simulink model "mdt_snap_10ch_daq"  (R2018a)
settings: Solver=VariableStepAuto  StartTime=0.0  StopTime=2000  RelTol=1e-3
libraries: xbsIndex_r4 x1064, xps_library x6, casper_library_misc x6, simulink x1
(part 1 of 12)
settings Model: Creator=aragorn  LastModifiedBy=aragorn

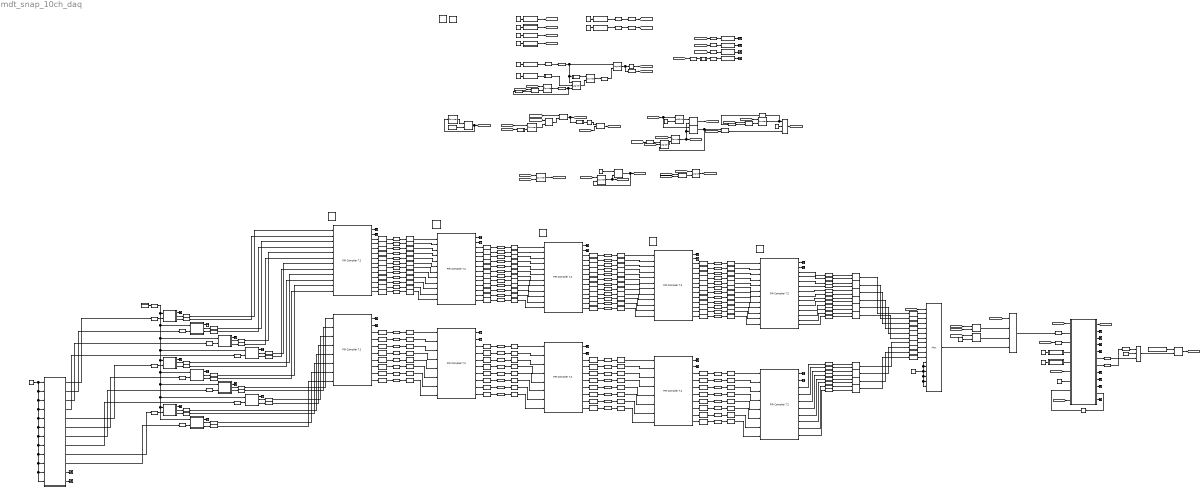
== system mdt_snap_10ch_daq ==
  note: Circuit to decimate FPGA clock. Decimation factor M stored as a constant.
      | Output: a high pulse 1 clock width at the last cycle of every M cycles.
      | Note: initial value of counter is 1; number of bits for counter and constant should be same or sufficient to accomodate value M.
  note: 1/1000 x FPGA clock period.
  note: stationIdx: MDT station ID
      |
      | snapIdx: SNAP board ID in the station
      |
      | Nelements: number of elements in instrument, i.e. number of analogue channels that the SNAP board need to process: at most 10.
      |
      | SperElement: number of samples taken per analogue channel to fit into 1 UDP packet.
      |
      | PktLimit: number of packets to acquire in one go and stored in bram.
  note: ch_valid is set to high after each decimated clk, during {0, Nelements-1}.
      | ch_last is 1 on clock cycle when counter = Nelements-1.
  note: Circuit counts the number of samples per channel being added to the current packet. Once the number of samples is equal to SperElement the end_pkt signal will be high at the last sample of the last batch in the packet. Then, on the next clock the new_pkt signal is high.
      | Note that the new_pkt signal is also set to high when enable pkt is set to 1 at the beginning of acquisition.
  note: Circuit to enable input of the header to the 10gbe block.
  note: Circuit to enable data input to the 10gbe block.
  note: Circuit to count packets for the duration of observation.
  note: 2^32 - 1 = 4294967295
  note: When enable_daq is set to 1, the packetiser will start working when the trigger for the 1PPS is received via 10 GbE from the script.
  note: Byte-swapping to obtain Little-Endian at output. Also concatenates the two samples to form a pair.
  note: SNAP FPGA is clocked at 250 MHz and ADC samples at 250 MSps. Therefore, we obtain 1 sample per analogue channel digitised.
      |
      | DDC mixer works with LO at 77.4 MHz and outputs complex samples.
      |
      | The 5-stage filter cuts out the relevant 250 kHz bandwidth centered at 327.4 MHz and decimates the sampling frequency to 250 kSps.
      |
      | The samples are then input sequentially to the 10gbe block. The packetiser circuit also includes a header with each packet.
  note: LPF with cut-off at 125 kHz and roll-off up to 250 kHz at -80 dB
      | Kaiser window with 82 taps.
      | Decimation factor: 4
      | Output at 500 kSps
  note: Quadrature mixing with LO at frequency = (10145/32768) x 250 MHz
      | = 77.4 MHz
  note: LPF with cut-off at 140 kHz and roll-off up to ~5 MHz at -98 dB
      | Kaiser window with 66 taps.
      | Decimation factor: 5
      | Output at 10 MSps
  note: LPF with cut-off at 130 kHz and roll-off up to 1 MHz at -89 dB
      | Kaiser window with 66 taps.
      | Decimation factor: 5
      | Output at 2 MSps
  note: LPF with cut-off at 123 kHz and roll-off up to 126 kHz at -72 dB
      | Kaiser window with 710 taps.
      | Decimation factor: 2
      | Output at 250 kSps
  note: LPF with cut-off at 140 kHz and roll-off up to ~25 MHz at -100 dB
      | Kaiser window with 66 taps.
      | Decimation factor: 5
      | Output at 50 MSps
  note: ADC2
      |
      | SMATP9
      | SMATP10
      | SMATP11
      | SMATP12
  note: SMATP1 -- SMATP6
  note: Decimation Filter Stage 1
  note: Digital Down-Conversion
  note: ADC
  note: SMATP7 -- SMATP10
  note: SMATP1 -- SMATP6
  note: SMATP7 -- SMATP10
  note: Decimation Filter Stage 2
  note: SMATP1 -- SMATP6
  note: SMATP7 -- SMATP10
  note: Decimation Filter Stage 3
  note: SMATP7 -- SMATP10
  note: SMATP1 -- SMATP6
  note: Decimation Filter Stage 4
  note: SMATP7 -- SMATP10
  note: SMATP1 -- SMATP6
  note: Decimation Filter Stage 5
  note: Byte-Swapping
  note: Packetisation
  note: Byte-swapping
      | for header
  note: LED 0 : data acquisition enabled
      |
      | LED 1 : 10 GbE port 0 is up and connected
      |
      | LED 2 : UDP packet being constructed
      |
      | LED 3 : end of current UDP packet
  note: ADC1
      |
      | SMATP5
      | SMATP6
      | SMATP7
      | SMATP8
  note: ADC0
      |
      | SMATP1
      | SMATP2
      | SMATP3
      | SMATP4
  note: Send data out in UDP packets
  note: Header
  note: Receive signal to start acquisition
  note: mdt_snap_10ch_daq.slx
      |
      | Copyright (c) 2020 Nitish Ragoomundun, Mauritius
      |
      | Permission is hereby granted, free of charge, to any person obtaining a copy
      | of this software and associated documentation files (the "Software"), to deal
      | in the Software without restriction, including without limitation the rights
      | to use, copy, modify, merge, publish, distribute, sublicense, and/or sell
      | copies of the Software, and to permit persons to whom the Software is
      | furnished to do so, subject to the following conditions:
      |
      | The above copyright notice and this permission notice shall be included in all
      | copies or substantial portions of the Software.
      |
      | THE SOFTWARE IS PROVIDED "AS IS", WITHOUT WARRANTY OF ANY KIND, EXPRESS OR
      | IMPLIED, INCLUDING BUT NOT LIMITED TO THE WARRANTIES OF MERCHANTABILITY,
      | FITNESS FOR A PARTICULAR PURPOSE AND NONINFRINGEMENT. IN NO EVENT SHALL THE
      | AUTHORS OR COPYRIGHT HOLDERS BE LIABLE FOR ANY CLAIM, DAMAGES OR OTHER
      | LIABILITY, WHETHER IN AN ACTION OF CONTRACT, TORT OR OTHERWISE, ARISING FROM,
      | OUT OF OR IN CONNECTION WITH THE SOFTWARE OR THE USE OR OTHER DEALINGS IN THE
      | SOFTWARE.
  " System Generator" : xbsIndex_r4/ System Generator  Tag=genX  xilinxfamily=kintex7  part=xc7k160t  speed=-2  package=ffg676  synthesis_tool=XST  clock_wrapper=Clock Enables  directory=/home/aragorn/Documents/SNAP/MDT_SNAP_DAQ/mdt_snap_10ch_daq/sysgen  proj_type=Vivado  Synth_file=Vivado Synthesis Defaults  Impl_file=Vivado Implementation Defaults  testbench=off  simulink_period=1  sysclk_period=4  dcm_input_clock_period=10  incr_netlist=off  trim_vbits=Everywhere in SubSystem  dbl_ovrd=According to Block Masks  core_generation=According to Block Masks  run_coregen=off  deprecated_control=off  eval_field=0  block_type=sysgen
  AddSub1 : xbsIndex_r4/AddSub  mode=Subtraction  use_carryin=off  use_carryout=off  en=off  latency=0  precision=User Defined  arith_type=Unsigned  n_bits=4  bin_pt=0  quantization=Truncate  overflow=Wrap  use_behavioral_HDL=off  hw_selection=Fabric  pipelined=off  dbl_ovrd=off  block_type=addsub
  Band-Limited White Noise : simulink/Sources/Band-Limited White Noise  Cov=[0.1]  Ts=1.0  seed=[23341]
  BitBasher{1..12} (12 alike) : xbsIndex_r4/BitBasher  bitexpr=c = {a[7:0], a[15:8], a[23:16], a[31:24], b[7:0], b[15:8], b[23:16], b[31:24]}  display_expr=off  sr_1=c  arith_type1=Unsigned  bin_pt1=0  sr_2=2  arith_type2=Unsigned  bin_pt2=0  sr_3=3  arith_type3=Unsigned  bin_pt3=0  sr_4=4  arith_type4=Unsigned  bin_pt4=0  dbl_ovrd=off  block_type=bitbasher
  Constant : xbsIndex_r4/Constant  const=1000  gui_display_data_type=Fixed-point  arith_type=Unsigned  n_bits=10  bin_pt=0  preci_type=Single  exp_width=8  frac_width=24  explicit_period=on  period=1  equ=P=C  opselect=C  inp2=PCIN>>17  opr=+  inp1=P  carry=CIN  dbl_ovrd=off  block_type=constant
  Constant{1..2,4,8,105..106,114} (7 alike) : Constant  Value=0
  Constant107 : xbsIndex_r4/Constant  const=0  gui_display_data_type=Fixed-point  arith_type=Unsigned  n_bits=32  bin_pt=0  preci_type=Single  exp_width=8  frac_width=24  explicit_period=on  period=1  equ=P=C  opselect=C  inp2=PCIN>>17  opr=+  inp1=P  carry=CIN  dbl_ovrd=off  block_type=constant
  Constant108 : Constant  Value=3
  Constant109 : Constant  Value=8
  Constant110 : xbsIndex_r4/Constant  const=1  gui_display_data_type=Fixed-point  arith_type=Unsigned  n_bits=1  bin_pt=0  preci_type=Single  exp_width=8  frac_width=24  explicit_period=on  period=1  equ=P=C  opselect=C  inp2=PCIN>>17  opr=+  inp1=P  carry=CIN  dbl_ovrd=off  block_type=constant
  Constant111 : xbsIndex_r4/Constant  const=0  gui_display_data_type=Boolean  arith_type=Boolean  n_bits=1  bin_pt=0  preci_type=Single  exp_width=8  frac_width=24  explicit_period=on  period=1  equ=P=C  opselect=C  inp2=PCIN>>17  opr=+  inp1=P  carry=CIN  dbl_ovrd=off  block_type=constant
  Constant3 : xbsIndex_r4/Constant  const=2  gui_display_data_type=Fixed-point  arith_type=Unsigned  n_bits=2  bin_pt=0  preci_type=Single  exp_width=8  frac_width=24  explicit_period=on  period=1  equ=P=C  opselect=C  inp2=PCIN>>17  opr=+  inp1=P  carry=CIN  dbl_ovrd=off  block_type=constant
  Constant5 : xbsIndex_r4/Constant  const=0  gui_display_data_type=Fixed-point  arith_type=Unsigned  n_bits=64  bin_pt=0  preci_type=Single  exp_width=8  frac_width=24  explicit_period=on  period=1  equ=P=C  opselect=C  inp2=PCIN>>17  opr=+  inp1=P  carry=CIN  dbl_ovrd=off  block_type=constant
  Constant6 : xbsIndex_r4/Constant  const=12012006508534266765  gui_display_data_type=Fixed-point  arith_type=Unsigned  n_bits=64  bin_pt=0  preci_type=Single  exp_width=8  frac_width=24  explicit_period=on  period=1  equ=P=C  opselect=C  inp2=PCIN>>17  opr=+  inp1=P  carry=CIN  dbl_ovrd=off  block_type=constant
  Constant7 : xbsIndex_r4/Constant  const=0  gui_display_data_type=Fixed-point  arith_type=Unsigned  n_bits=64  bin_pt=0  preci_type=Single  exp_width=8  frac_width=24  explicit_period=on  period=1  equ=P=C  opselect=C  inp2=PCIN>>17  opr=+  inp1=P  carry=CIN  dbl_ovrd=off  block_type=constant
  Constant9 : xbsIndex_r4/Constant  const=1  gui_display_data_type=Boolean  arith_type=Boolean  n_bits=16  bin_pt=14  preci_type=Single  exp_width=8  frac_width=24  explicit_period=on  period=1  equ=P=C  opselect=C  inp2=PCIN>>17  opr=+  inp1=P  carry=CIN  dbl_ovrd=off  block_type=constant
  Convert{,2,4,6,8..9,25..34,39..42} (20 alike) : xbsIndex_r4/Convert  gui_display_data_type=Fixed-point  arith_type="Signed  (2's comp)"  n_bits=16  bin_pt=12  float_type=Single  exp_bits=8  fraction_bits=24  quantization="Round  (unbiased: +/- Inf)"  overflow=Wrap  en=off  latency=1  pipeline=on  dbl_ovrd=off  block_type=convert
  Convert1 : xbsIndex_r4/Convert  gui_display_data_type=Boolean  arith_type=Boolean  n_bits=16  bin_pt=14  float_type=Single  exp_bits=8  fraction_bits=24  quantization=Truncate  overflow=Wrap  en=off  latency=0  pipeline=off  dbl_ovrd=off  block_type=convert
  Convert{10..15,43..56} (20 alike) : xbsIndex_r4/Convert  gui_display_data_type=Fixed-point  arith_type="Signed  (2's comp)"  n_bits=16  bin_pt=10  float_type=Single  exp_bits=8  fraction_bits=24  quantization="Round  (unbiased: +/- Inf)"  overflow=Wrap  en=off  latency=1  pipeline=on  dbl_ovrd=off  block_type=convert
  Convert{3,16..20,61..73,78} (20 alike) : xbsIndex_r4/Convert  gui_display_data_type=Fixed-point  arith_type="Signed  (2's comp)"  n_bits=16  bin_pt=8  float_type=Single  exp_bits=8  fraction_bits=24  quantization="Round  (unbiased: +/- Inf)"  overflow=Wrap  en=off  latency=1  pipeline=on  dbl_ovrd=off  block_type=convert
  Convert{5,7,21..24,79..90,95..96} (20 alike) : xbsIndex_r4/Convert  gui_display_data_type=Fixed-point  arith_type="Signed  (2's comp)"  n_bits=16  bin_pt=6  float_type=Single  exp_bits=8  fraction_bits=24  quantization="Round  (unbiased: +/- Inf)"  overflow=Wrap  en=off  latency=1  pipeline=on  dbl_ovrd=off  block_type=convert
  Counter1 : xbsIndex_r4/Counter  cnt_type=Free Running  cnt_to=Inf  operation=Up  start_count=0  cnt_by_val=1  arith_type=Unsigned  n_bits=2  bin_pt=0  load_pin=off  rst=on  en=on  explicit_period=on  period=1  use_behavioral_HDL=off  implementation=Fabric  dbl_ovrd=off  block_type=counter
  Counter10 : xbsIndex_r4/Counter  cnt_type=Free Running  cnt_to=Inf  operation=Up  start_count=0  cnt_by_val=1  arith_type=Unsigned  n_bits=16  bin_pt=0  load_pin=off  rst=on  en=on  explicit_period=on  period=1  use_behavioral_HDL=off  implementation=Fabric  dbl_ovrd=off  block_type=counter
  Counter11 : xbsIndex_r4/Counter  cnt_type=Free Running  cnt_to=Inf  operation=Up  start_count=0  cnt_by_val=1  arith_type=Unsigned  n_bits=1  bin_pt=0  load_pin=off  rst=on  en=on  explicit_period=on  period=1  use_behavioral_HDL=off  implementation=Fabric  dbl_ovrd=off  block_type=counter
  Counter2 : xbsIndex_r4/Counter  cnt_type=Free Running  cnt_to=Inf  operation=Up  start_count=0  cnt_by_val=1  arith_type=Unsigned  n_bits=32  bin_pt=0  load_pin=off  rst=on  en=on  explicit_period=on  period=1  use_behavioral_HDL=off  implementation=Fabric  dbl_ovrd=off  block_type=counter
  Counter3 : xbsIndex_r4/Counter  cnt_type=Free Running  cnt_to=Inf  operation=Up  start_count=1  cnt_by_val=1  arith_type=Unsigned  n_bits=10  bin_pt=0  load_pin=off  rst=on  en=off  explicit_period=on  period=1  use_behavioral_HDL=off  implementation=Fabric  dbl_ovrd=off  block_type=counter
  Counter4 : xbsIndex_r4/Counter  cnt_type=Free Running  cnt_to=Inf  operation=Up  start_count=0  cnt_by_val=1  arith_type=Unsigned  n_bits=2  bin_pt=0  load_pin=off  rst=on  en=on  explicit_period=on  period=1  use_behavioral_HDL=off  implementation=Fabric  dbl_ovrd=off  block_type=counter
  Counter6 : xbsIndex_r4/Counter  cnt_type=Free Running  cnt_to=Inf  operation=Up  start_count=0  cnt_by_val=1  arith_type=Unsigned  n_bits=2  bin_pt=0  load_pin=off  rst=on  en=on  explicit_period=on  period=1  use_behavioral_HDL=off  implementation=Fabric  dbl_ovrd=off  block_type=counter
  Counter7 : xbsIndex_r4/Counter  cnt_type=Free Running  cnt_to=Inf  operation=Up  start_count=0  cnt_by_val=1  arith_type=Unsigned  n_bits=4  bin_pt=0  load_pin=off  rst=on  en=on  explicit_period=on  period=1  use_behavioral_HDL=off  implementation=Fabric  dbl_ovrd=off  block_type=counter
  Delay1 : xbsIndex_r4/Delay  rst=off  infoeditControl=Selection of Reset will increase slice count due to use of real FFs and instead of SRLs  en=off  latency=1  reg_retiming=off  dbl_ovrd=off  block_type=delay
  Delay2 : xbsIndex_r4/Delay  rst=off  infoeditControl=Selection of Reset will increase slice count due to use of real FFs and instead of SRLs  en=off  latency=1  reg_retiming=off  dbl_ovrd=off  block_type=delay
  Delay4 : xbsIndex_r4/Delay  rst=off  infoeditControl=Selection of Reset will increase slice count due to use of real FFs and instead of SRLs  en=off  latency=1  reg_retiming=off  dbl_ovrd=off  block_type=delay
  Inverter1 : xbsIndex_r4/Inverter  en=off  latency=0  dbl_ovrd=off  block_type=inv
  Inverter2 : xbsIndex_r4/Inverter  en=off  latency=0  dbl_ovrd=off  block_type=inv
  Inverter3 : xbsIndex_r4/Inverter  en=off  latency=0  dbl_ovrd=off  block_type=inv
  Logical1 : xbsIndex_r4/Logical  logical_function=AND  inputs=3  en=off  latency=0  precision=User Defined  arith_type=Boolean  n_bits=1  bin_pt=0  align_bp=on  dbl_ovrd=off  block_type=logical
  Logical10 : xbsIndex_r4/Logical  logical_function=OR  inputs=2  en=off  latency=0  precision=User Defined  arith_type=Boolean  n_bits=1  bin_pt=0  align_bp=on  dbl_ovrd=off  block_type=logical
  Logical{2..3,6..9} (6 alike) : xbsIndex_r4/Logical  logical_function=AND  inputs=2  en=off  latency=0  precision=User Defined  arith_type=Boolean  n_bits=1  bin_pt=0  align_bp=on  dbl_ovrd=off  block_type=logical
  Logical4 : xbsIndex_r4/Logical  logical_function=OR  inputs=2  en=off  latency=0  precision=User Defined  arith_type=Boolean  n_bits=1  bin_pt=0  align_bp=on  dbl_ovrd=off  block_type=logical
  Logical5 : xbsIndex_r4/Logical  logical_function=AND  inputs=3  en=off  latency=0  precision=User Defined  arith_type=Boolean  n_bits=1  bin_pt=0  align_bp=on  dbl_ovrd=off  block_type=logical
  Mux1 : xbsIndex_r4/Mux  inputs=2  en=off  latency=0  precision=Full  arith_type=Unsigned  n_bits=16  bin_pt=14  quantization=Truncate  overflow=Wrap  dbl_ovrd=off  block_type=mux
  Mux3 : xbsIndex_r4/Mux  inputs=16  en=off  latency=0  precision=Full  arith_type=Unsigned  n_bits=16  bin_pt=14  quantization=Truncate  overflow=Wrap  dbl_ovrd=off  block_type=mux
  Mux4 : xbsIndex_r4/Mux  inputs=3  en=off  latency=0  precision=Full  arith_type=Unsigned  n_bits=16  bin_pt=14  quantization=Truncate  overflow=Wrap  dbl_ovrd=off  block_type=mux
  Mux5 : xbsIndex_r4/Mux  inputs=2  en=off  latency=0  precision=Full  arith_type=Unsigned  n_bits=16  bin_pt=14  quantization=Truncate  overflow=Wrap  dbl_ovrd=off  block_type=mux
  Nelements : Subsystem  Tag=xps:sw_reg  AncestorBlock=xps_library/Memory/software_register  mask(swreg){io_dir=From Processor, io_delay=0, init_val=0, sample_period=1, names=reg, bitwidths=32, bin_pts=0, arith_types=0, sim_port=on, show_format=on}
      mask prompts: io_dir "I/O direction"; io_delay "I/O delay"; init_val "Initial Value"; sample_period "Sample period"; names "Bitfield names [msb...lsb]"; bitwidths "Bitfield widths"; bin_pts "Bitfield binary pts"; arith_types "Bitfield types, ufix=0, fix=1, bool=2"; sim_port "Provide sim input/output?"; show_format "Print format string?"
      mask help: A 32-bit software-accessible register. Can be divided into bitfields of varying widths and types using the fields in the block mask.
      mask init:
      | swreg_init(gcb)
      settings: AttributesFormatString=1input:uf32.0 = 32 bits
      mask TypeOptions io_dir: To Processor | From Processor
      mask Callback io_dir:
      | mask_enables = get_param(gcb, 'MaskEnables');
      | mask_names = get_param(gcb, 'MaskNames');
      | if strcmp(get_param(gcb, 'io_dir'), 'To Processor'),
      |     mask_enables{ismember(mask_names, 'sample_period')} = 'off';
      | else
      |     mask_enables{ismember(mask_names, 'sample_period')} = 'on';
      | end
      | set_param(gcb, 'MaskEnables', mask_enables);
      mask DialogControl ParameterTabVar0 Prompt: Setup
  Pulse Generator : DiscretePulseGenerator  PulseType=Time based  Period=1  PulseWidth=20
  Register{1..32,38..42,44..48,55} (43 alike) : xbsIndex_r4/Register  init=0  rst=off  en=off  dbl_ovrd=off  block_type=register
  Reinterpret{1..6,25,107..115,120..124} (21 alike) : xbsIndex_r4/Reinterpret  force_arith_type=on  arith_type=Unsigned  force_bin_pt=on  bin_pt=0  block_type=reinterpret
  Reinterpret{7..11,36,89..99,101,103..104} (20 alike) : xbsIndex_r4/Reinterpret  force_arith_type=off  arith_type=Unsigned  force_bin_pt=on  bin_pt=22  block_type=reinterpret
  Reinterpret{12..24,29..31,33..34,51..52} (20 alike) : xbsIndex_r4/Reinterpret  force_arith_type=off  arith_type=Unsigned  force_bin_pt=on  bin_pt=28  block_type=reinterpret
  Reinterpret{32,45..49,71..84} (20 alike) : xbsIndex_r4/Reinterpret  force_arith_type=off  arith_type=Unsigned  force_bin_pt=on  bin_pt=24  block_type=reinterpret
  Reinterpret{37,40..44,53..66} (20 alike) : xbsIndex_r4/Reinterpret  force_arith_type=off  arith_type=Unsigned  force_bin_pt=on  bin_pt=26  block_type=reinterpret
  Relational{1..2,10,13} (4 alike) : xbsIndex_r4/Relational  mode=a=b  op_type=Bool  en=off  latency=0  dbl_ovrd=off  block_type=relational
  Relational11 : xbsIndex_r4/Relational  mode=a>b  op_type=Bool  en=off  latency=0  dbl_ovrd=off  block_type=relational
  Relational12 : xbsIndex_r4/Relational  mode=a>b  op_type=Bool  en=off  latency=0  dbl_ovrd=off  block_type=relational
  SNAP : xps_library/Platforms/SNAP  Tag=xps:xsg  hw_sys=SNAP:xc7k160t  clk_src=adc0_clk  clk_rate=250  use_microblaze=off  sample_period=1  synthesis_tool=XST
      settings: SourceProductName=CASPER XPS Blockset
  Shift{,1..32,37..54,59..72,76,78..90,95} (80 alike) : xbsIndex_r4/Shift  shift_dir=Left  shift_bits=2  en=off  latency=1  precision=Full  arith_type="Signed  (2's comp)"  n_bits=16  bin_pt=14  quantization=Truncate  overflow=Wrap  dbl_ovrd=off  block_type=shift
  Slice{1..5} (5 alike) : xbsIndex_r4/Slice  nbits=1  boolean_output=on  mode=Lower Bit Location + Width  bit1=0  base1=MSB of Input  bit0=0  base0=LSB of Input  dbl_ovrd=off  block_type=slice
  SperElement : Subsystem  Tag=xps:sw_reg  AncestorBlock=xps_library/Memory/software_register  mask(swreg){io_dir=From Processor, io_delay=0, init_val=0, sample_period=1, names=reg, bitwidths=32, bin_pts=0, arith_types=0, sim_port=on, show_format=on}
      mask prompts: io_dir "I/O direction"; io_delay "I/O delay"; init_val "Initial Value"; sample_period "Sample period"; names "Bitfield names [msb...lsb]"; bitwidths "Bitfield widths"; bin_pts "Bitfield binary pts"; arith_types "Bitfield types, ufix=0, fix=1, bool=2"; sim_port "Provide sim input/output?"; show_format "Print format string?"
      mask help: A 32-bit software-accessible register. Can be divided into bitfields of varying widths and types using the fields in the block mask.
      mask init:
      | swreg_init(gcb)
      settings: AttributesFormatString=1input:uf32.0 = 32 bits
      mask TypeOptions io_dir: To Processor | From Processor
      mask Callback io_dir:
      | mask_enables = get_param(gcb, 'MaskEnables');
      | mask_names = get_param(gcb, 'MaskNames');
      | if strcmp(get_param(gcb, 'io_dir'), 'To Processor'),
      |     mask_enables{ismember(mask_names, 'sample_period')} = 'off';
      | else
      |     mask_enables{ismember(mask_names, 'sample_period')} = 'on';
      | end
      | set_param(gcb, 'MaskEnables', mask_enables);
      mask DialogControl ParameterTabVar0 Prompt: Setup
  Stage1_ch1-6 : xbsIndex_r4/FIR Compiler 7.2   coefficientvector=[-0.000002449538004038990423916243369117, -0.000005500349966184503970535908667915, -0.000005285271766498275070804251096756, 0.000005201883925181383781951010430999, 0.000035996819259535929092820583097278, 0.000098266946066012054311622492264177, 0.000200426952388683672721253481441294, 0.000342426747931809155513910303270108, 0.000509090254199270376977981555910446, 0.000664151073096023460660963788626531, 0.000747226168430985336448013622856478, 0.000676147634572773440636561659289327, 0.000356634720256595130240262481180479, -0.000299853285296282356942043634262518, -0.001351005061725356337642978132862481, -0.002794317437538150830644845257211272, -0.004538578190165965149660554089905417, -0.006382626815274574164082999061520240, -0.008008145384657154586260929818308795, -0.008992087975882372477554049794434831, -0.008841716737080985988317394230762147, -0.007051359492092778950833587003899083, -0.003175552799073219373965359935141350, 0.003090960705163858963928635859019777, 0.011838921151523604941013800839755276, 0.022889486804945475412198518938566849, 0.035770526437351526927166389668855117, 0.049732447110816674351596589076507370, 0.063805828276941325971627350099879549, 0.076896215021160799207855518488941015, 0.087904748254232167870014791333233006, 0.095858174396951711937475693048327229, 0.100029250702665883920872147427871823, 0.100029250702665883920872147427871823, 0.095858174396951711937475693048327229, 0.087904748254232167870014791333233006, 0.076896215021160799207855518488941015, 0.063805828276941325971627350099879549, 0.049732447110816674351596589076507370, 0.035770526437351526927166389668855117, 0.022889486804945475412198518938566849, 0.011838921151523604941013800839755276, 0.003090960705163858963928635859019777, -0.003175552799073219373965359935141350, -0.007051359492092778950833587003899083, -0.008841716737080985988317394230762147, -0.008992087975882372477554049794434831, -0.008008145384657154586260929818308795, -0.006382626815274574164082999061520240, -0.004538578190165965149660554089905417, -0.002794317437538150830644845257211272, -0.001351005061725356337642978132862481, -0.000299853285296282356942043634262518, 0.000356634720256595130240262481180479, 0.000676147634572773440636561659289327, 0.000747226168430985336448013622856478, 0.000664151073096023460660963788626531, 0.000509090254199270376977981555910446, 0.000342426747931809155513910303270108, 0.000200426952388683672721253481441294, 0.000098266946066012054311622492264177, 0.000035996819259535929092820583097278, 0.000005201883925181383781951010430999, -0.000005285271766498275070804251096756, -0.000005500349966184503970535908667915, -0.000002449538004038990423916243369117]  coefficient_sets=1  coefficient_reload=off  filter_type=Decimation  rate_change_type=Integer  interpolation_rate=1  decimation_rate=5  zero_pack_factor=1  channel_sequence=Basic  number_channels=1  pattern_list='P4-0,P4-1,P4-2,P4-3,P4-4'  number_paths=12  ratespecification=Maximum_Possible  sampleperiod=1  hardwareoversamplingrate=1  coefficient_sign=Signed  quantization=Maximize_Dynamic_Range  coefficient_width=25  bestprecision=off  coefficient_fractional_bits=24  coefficient_structure=Inferred  output_rounding_mode=Symmetric_Rounding_to_Infinity  output_width=32  filter_architecture=Systolic_Multiply_Accumulate  optimization_goal=Area  optimization_list='None'  data_buffer_type=Automatic  coefficient_buffer_type=Automatic  input_buffer_type=Automatic  output_buffer_type=Automatic  preference_for_other_storage=Automatic  multi_column_support=Automatic  columnconfig='7'  inter_column_pipe_length=4  data_has_tlast=Not_Required  m_data_has_tready=off  s_data_has_fifo=off  s_data_has_tuser=Not_Required  m_data_has_tuser=Not_Required  s_config_sync_mode=On_Vector  s_config_method=Single  num_reload_slots=1  has_aclken=off  has_aresetn=off  infoeditControl=ARESETn must be asserted for a minimum of 2 cycles  reset_data_vector=on  trim_axipin_name=on  simulation_type=hybrid_sim  simulation_model=sysgen:xfirv7_2_cmodel  data_path_portlist={ 's_axis_data_tdata', 'm_axis_data_tdata' }  passband_min=0.0  passband_max=0.5  stopband_min=0.5  stopband_max=1.0  filter_selection=1  gui_behaviour='Sysgen_GUI'  data_sign=Signed  data_width=16  data_fractional_bits=0  data_tuser_width=1  wrapper_available=true  ip_wrap_arbitrary_binary_point=true  ip_name=FIR Compiler  ip_version=7.2  dsptool_ready=true  ipcore_usecache=true  ipcore_useipmodelcache=true  port_translation_map={ 'aclken' => 'en', 'aresetn' => 'rst' }  run_core_at_system_period=true  ipcore_xco_need_fpga_part=true  block_type=fir_compiler_v7_2
      settings: infoedit=Maximum Possible : Maximizes oversampling rate. Abstracted input handshake (no s_data_tvalid) and automatic rate propagation.<br>Hardware Oversampling Rate : Specifies oversampling rate relative to the input sample period. Abstracted input handshake (no s_data_tvalid) and automatic rate propagation.<br>Input/Output Sample Period : Specifies absolute oversampling rate. No input handshake abstraction (exposes s_data_tvalid) and no rate propagation.
  Stage1_ch7-10 : xbsIndex_r4/FIR Compiler 7.2   coefficientvector=[-0.000002449538004038990423916243369117, -0.000005500349966184503970535908667915, -0.000005285271766498275070804251096756, 0.000005201883925181383781951010430999, 0.000035996819259535929092820583097278, 0.000098266946066012054311622492264177, 0.000200426952388683672721253481441294, 0.000342426747931809155513910303270108, 0.000509090254199270376977981555910446, 0.000664151073096023460660963788626531, 0.000747226168430985336448013622856478, 0.000676147634572773440636561659289327, 0.000356634720256595130240262481180479, -0.000299853285296282356942043634262518, -0.001351005061725356337642978132862481, -0.002794317437538150830644845257211272, -0.004538578190165965149660554089905417, -0.006382626815274574164082999061520240, -0.008008145384657154586260929818308795, -0.008992087975882372477554049794434831, -0.008841716737080985988317394230762147, -0.007051359492092778950833587003899083, -0.003175552799073219373965359935141350, 0.003090960705163858963928635859019777, 0.011838921151523604941013800839755276, 0.022889486804945475412198518938566849, 0.035770526437351526927166389668855117, 0.049732447110816674351596589076507370, 0.063805828276941325971627350099879549, 0.076896215021160799207855518488941015, 0.087904748254232167870014791333233006, 0.095858174396951711937475693048327229, 0.100029250702665883920872147427871823, 0.100029250702665883920872147427871823, 0.095858174396951711937475693048327229, 0.087904748254232167870014791333233006, 0.076896215021160799207855518488941015, 0.063805828276941325971627350099879549, 0.049732447110816674351596589076507370, 0.035770526437351526927166389668855117, 0.022889486804945475412198518938566849, 0.011838921151523604941013800839755276, 0.003090960705163858963928635859019777, -0.003175552799073219373965359935141350, -0.007051359492092778950833587003899083, -0.008841716737080985988317394230762147, -0.008992087975882372477554049794434831, -0.008008145384657154586260929818308795, -0.006382626815274574164082999061520240, -0.004538578190165965149660554089905417, -0.002794317437538150830644845257211272, -0.001351005061725356337642978132862481, -0.000299853285296282356942043634262518, 0.000356634720256595130240262481180479, 0.000676147634572773440636561659289327, 0.000747226168430985336448013622856478, 0.000664151073096023460660963788626531, 0.000509090254199270376977981555910446, 0.000342426747931809155513910303270108, 0.000200426952388683672721253481441294, 0.000098266946066012054311622492264177, 0.000035996819259535929092820583097278, 0.000005201883925181383781951010430999, -0.000005285271766498275070804251096756, -0.000005500349966184503970535908667915, -0.000002449538004038990423916243369117]  coefficient_sets=1  coefficient_reload=off  filter_type=Decimation  rate_change_type=Integer  interpolation_rate=1  decimation_rate=5  zero_pack_factor=1  channel_sequence=Basic  number_channels=1  pattern_list='P4-0,P4-1,P4-2,P4-3,P4-4'  number_paths=8  ratespecification=Maximum_Possible  sampleperiod=1  hardwareoversamplingrate=1  coefficient_sign=Signed  quantization=Maximize_Dynamic_Range  coefficient_width=25  bestprecision=off  coefficient_fractional_bits=24  coefficient_structure=Inferred  output_rounding_mode=Symmetric_Rounding_to_Infinity  output_width=32  filter_architecture=Systolic_Multiply_Accumulate  optimization_goal=Area  optimization_list='None'  data_buffer_type=Automatic  coefficient_buffer_type=Automatic  input_buffer_type=Automatic  output_buffer_type=Automatic  preference_for_other_storage=Automatic  multi_column_support=Automatic  columnconfig='7'  inter_column_pipe_length=4  data_has_tlast=Not_Required  m_data_has_tready=off  s_data_has_fifo=off  s_data_has_tuser=Not_Required  m_data_has_tuser=Not_Required  s_config_sync_mode=On_Vector  s_config_method=Single  num_reload_slots=1  has_aclken=off  has_aresetn=off  infoeditControl=ARESETn must be asserted for a minimum of 2 cycles  reset_data_vector=on  trim_axipin_name=on  simulation_type=hybrid_sim  simulation_model=sysgen:xfirv7_2_cmodel  data_path_portlist={ 's_axis_data_tdata', 'm_axis_data_tdata' }  passband_min=0.0  passband_max=0.5  stopband_min=0.5  stopband_max=1.0  filter_selection=1  gui_behaviour='Sysgen_GUI'  data_sign=Signed  data_width=16  data_fractional_bits=0  data_tuser_width=1  wrapper_available=true  ip_wrap_arbitrary_binary_point=true  ip_name=FIR Compiler  ip_version=7.2  dsptool_ready=true  ipcore_usecache=true  ipcore_useipmodelcache=true  port_translation_map={ 'aclken' => 'en', 'aresetn' => 'rst' }  run_core_at_system_period=true  ipcore_xco_need_fpga_part=true  block_type=fir_compiler_v7_2
      settings: infoedit=Maximum Possible : Maximizes oversampling rate. Abstracted input handshake (no s_data_tvalid) and automatic rate propagation.<br>Hardware Oversampling Rate : Specifies oversampling rate relative to the input sample period. Abstracted input handshake (no s_data_tvalid) and automatic rate propagation.<br>Input/Output Sample Period : Specifies absolute oversampling rate. No input handshake abstraction (exposes s_data_tvalid) and no rate propagation.
  Stage1_design : xbsIndex_r4/FDATool  block_type=fdatool
      settings: infoedit=FDATool
  Stage2_ch1-6 : xbsIndex_r4/FIR Compiler 7.2   coefficientvector=[-0.000003550691476594369524425343770390, -0.000008806083736990591198830202745995, -0.000012056289802994472735607131563817, -0.000005760556923833457625952394337565, 0.000021610725434097651225396480301199, 0.000083839678980122961252444135915595, 0.000192931647551063497518855638368506, 0.000352842073664228763566624857972442, 0.000551815424117022739272653275577340, 0.000755086825918051371582528918935395, 0.000900432827153620392313104758841291, 0.000899352585708945609192788150920705, 0.000646272917823731657231689506915017, 0.000036980443112204448906452786127729, -0.001004438412821170986330421293075687, -0.002493234695150796289414563133846058, -0.004351623589594994130635985385424646, -0.006383508642219052654775968136391384, -0.008263905619471481264759482598947215, -0.009549559959545423151738852141079405, -0.009714446432164439496070862389842659, -0.008209625876054615911669998240540735, -0.004541980071994147771796690449264133, 0.001638398816034949793951636110023173, 0.010455874012147550744522561672056326, 0.021747002079171434685278541110164951, 0.035031921910781811668744722965129767, 0.049528746177353505375506870223034638, 0.064213832055059982817368791074841283, 0.077923150644354163829596870982641121, 0.089482532970763140056646989251021295, 0.097848801913986011014046084710571449, 0.102240912741978245970031480283068958, 0.102240912741978245970031480283068958, 0.097848801913986011014046084710571449, 0.089482532970763140056646989251021295, 0.077923150644354163829596870982641121, 0.064213832055059982817368791074841283, 0.049528746177353505375506870223034638, 0.035031921910781811668744722965129767, 0.021747002079171434685278541110164951, 0.010455874012147550744522561672056326, 0.001638398816034949793951636110023173, -0.004541980071994147771796690449264133, -0.008209625876054615911669998240540735, -0.009714446432164439496070862389842659, -0.009549559959545423151738852141079405, -0.008263905619471481264759482598947215, -0.006383508642219052654775968136391384, -0.004351623589594994130635985385424646, -0.002493234695150796289414563133846058, -0.001004438412821170986330421293075687, 0.000036980443112204448906452786127729, 0.000646272917823731657231689506915017, 0.000899352585708945609192788150920705, 0.000900432827153620392313104758841291, 0.000755086825918051371582528918935395, 0.000551815424117022739272653275577340, 0.000352842073664228763566624857972442, 0.000192931647551063497518855638368506, 0.000083839678980122961252444135915595, 0.000021610725434097651225396480301199, -0.000005760556923833457625952394337565, -0.000012056289802994472735607131563817, -0.000008806083736990591198830202745995, -0.000003550691476594369524425343770390]  coefficient_sets=1  coefficient_reload=off  filter_type=Decimation  rate_change_type=Integer  interpolation_rate=1  decimation_rate=5  zero_pack_factor=1  channel_sequence=Basic  number_channels=1  pattern_list='P4-0,P4-1,P4-2,P4-3,P4-4'  number_paths=12  ratespecification=Maximum_Possible  sampleperiod=1  hardwareoversamplingrate=1  coefficient_sign=Signed  quantization=Maximize_Dynamic_Range  coefficient_width=25  bestprecision=off  coefficient_fractional_bits=24  coefficient_structure=Inferred  output_rounding_mode=Symmetric_Rounding_to_Infinity  output_width=32  filter_architecture=Systolic_Multiply_Accumulate  optimization_goal=Area  optimization_list='None'  data_buffer_type=Automatic  coefficient_buffer_type=Automatic  input_buffer_type=Automatic  output_buffer_type=Automatic  preference_for_other_storage=Automatic  multi_column_support=Automatic  columnconfig='7'  inter_column_pipe_length=4  data_has_tlast=Not_Required  m_data_has_tready=off  s_data_has_fifo=off  s_data_has_tuser=Not_Required  m_data_has_tuser=Not_Required  s_config_sync_mode=On_Vector  s_config_method=Single  num_reload_slots=1  has_aclken=off  has_aresetn=off  infoeditControl=ARESETn must be asserted for a minimum of 2 cycles  reset_data_vector=on  trim_axipin_name=on  simulation_type=hybrid_sim  simulation_model=sysgen:xfirv7_2_cmodel  data_path_portlist={ 's_axis_data_tdata', 'm_axis_data_tdata' }  passband_min=0.0  passband_max=0.5  stopband_min=0.5  stopband_max=1.0  filter_selection=1  gui_behaviour='Sysgen_GUI'  data_sign=Signed  data_width=16  data_fractional_bits=0  data_tuser_width=1  wrapper_available=true  ip_wrap_arbitrary_binary_point=true  ip_name=FIR Compiler  ip_version=7.2  dsptool_ready=true  ipcore_usecache=true  ipcore_useipmodelcache=true  port_translation_map={ 'aclken' => 'en', 'aresetn' => 'rst' }  run_core_at_system_period=true  ipcore_xco_need_fpga_part=true  block_type=fir_compiler_v7_2
      settings: infoedit=Maximum Possible : Maximizes oversampling rate. Abstracted input handshake (no s_data_tvalid) and automatic rate propagation.<br>Hardware Oversampling Rate : Specifies oversampling rate relative to the input sample period. Abstracted input handshake (no s_data_tvalid) and automatic rate propagation.<br>Input/Output Sample Period : Specifies absolute oversampling rate. No input handshake abstraction (exposes s_data_tvalid) and no rate propagation.
  Stage2_ch7-10 : xbsIndex_r4/FIR Compiler 7.2   coefficientvector=[-0.000003550691476594369524425343770390, -0.000008806083736990591198830202745995, -0.000012056289802994472735607131563817, -0.000005760556923833457625952394337565, 0.000021610725434097651225396480301199, 0.000083839678980122961252444135915595, 0.000192931647551063497518855638368506, 0.000352842073664228763566624857972442, 0.000551815424117022739272653275577340, 0.000755086825918051371582528918935395, 0.000900432827153620392313104758841291, 0.000899352585708945609192788150920705, 0.000646272917823731657231689506915017, 0.000036980443112204448906452786127729, -0.001004438412821170986330421293075687, -0.002493234695150796289414563133846058, -0.004351623589594994130635985385424646, -0.006383508642219052654775968136391384, -0.008263905619471481264759482598947215, -0.009549559959545423151738852141079405, -0.009714446432164439496070862389842659, -0.008209625876054615911669998240540735, -0.004541980071994147771796690449264133, 0.001638398816034949793951636110023173, 0.010455874012147550744522561672056326, 0.021747002079171434685278541110164951, 0.035031921910781811668744722965129767, 0.049528746177353505375506870223034638, 0.064213832055059982817368791074841283, 0.077923150644354163829596870982641121, 0.089482532970763140056646989251021295, 0.097848801913986011014046084710571449, 0.102240912741978245970031480283068958, 0.102240912741978245970031480283068958, 0.097848801913986011014046084710571449, 0.089482532970763140056646989251021295, 0.077923150644354163829596870982641121, 0.064213832055059982817368791074841283, 0.049528746177353505375506870223034638, 0.035031921910781811668744722965129767, 0.021747002079171434685278541110164951, 0.010455874012147550744522561672056326, 0.001638398816034949793951636110023173, -0.004541980071994147771796690449264133, -0.008209625876054615911669998240540735, -0.009714446432164439496070862389842659, -0.009549559959545423151738852141079405, -0.008263905619471481264759482598947215, -0.006383508642219052654775968136391384, -0.004351623589594994130635985385424646, -0.002493234695150796289414563133846058, -0.001004438412821170986330421293075687, 0.000036980443112204448906452786127729, 0.000646272917823731657231689506915017, 0.000899352585708945609192788150920705, 0.000900432827153620392313104758841291, 0.000755086825918051371582528918935395, 0.000551815424117022739272653275577340, 0.000352842073664228763566624857972442, 0.000192931647551063497518855638368506, 0.000083839678980122961252444135915595, 0.000021610725434097651225396480301199, -0.000005760556923833457625952394337565, -0.000012056289802994472735607131563817, -0.000008806083736990591198830202745995, -0.000003550691476594369524425343770390]  coefficient_sets=1  coefficient_reload=off  filter_type=Decimation  rate_change_type=Integer  interpolation_rate=1  decimation_rate=5  zero_pack_factor=1  channel_sequence=Basic  number_channels=1  pattern_list='P4-0,P4-1,P4-2,P4-3,P4-4'  number_paths=8  ratespecification=Maximum_Possible  sampleperiod=1  hardwareoversamplingrate=1  coefficient_sign=Signed  quantization=Maximize_Dynamic_Range  coefficient_width=25  bestprecision=off  coefficient_fractional_bits=24  coefficient_structure=Inferred  output_rounding_mode=Symmetric_Rounding_to_Infinity  output_width=32  filter_architecture=Systolic_Multiply_Accumulate  optimization_goal=Area  optimization_list='None'  data_buffer_type=Automatic  coefficient_buffer_type=Automatic  input_buffer_type=Automatic  output_buffer_type=Automatic  preference_for_other_storage=Automatic  multi_column_support=Automatic  columnconfig='7'  inter_column_pipe_length=4  data_has_tlast=Not_Required  m_data_has_tready=off  s_data_has_fifo=off  s_data_has_tuser=Not_Required  m_data_has_tuser=Not_Required  s_config_sync_mode=On_Vector  s_config_method=Single  num_reload_slots=1  has_aclken=off  has_aresetn=off  infoeditControl=ARESETn must be asserted for a minimum of 2 cycles  reset_data_vector=on  trim_axipin_name=on  simulation_type=hybrid_sim  simulation_model=sysgen:xfirv7_2_cmodel  data_path_portlist={ 's_axis_data_tdata', 'm_axis_data_tdata' }  passband_min=0.0  passband_max=0.5  stopband_min=0.5  stopband_max=1.0  filter_selection=1  gui_behaviour='Sysgen_GUI'  data_sign=Signed  data_width=16  data_fractional_bits=0  data_tuser_width=1  wrapper_available=true  ip_wrap_arbitrary_binary_point=true  ip_name=FIR Compiler  ip_version=7.2  dsptool_ready=true  ipcore_usecache=true  ipcore_useipmodelcache=true  port_translation_map={ 'aclken' => 'en', 'aresetn' => 'rst' }  run_core_at_system_period=true  ipcore_xco_need_fpga_part=true  block_type=fir_compiler_v7_2
      settings: infoedit=Maximum Possible : Maximizes oversampling rate. Abstracted input handshake (no s_data_tvalid) and automatic rate propagation.<br>Hardware Oversampling Rate : Specifies oversampling rate relative to the input sample period. Abstracted input handshake (no s_data_tvalid) and automatic rate propagation.<br>Input/Output Sample Period : Specifies absolute oversampling rate. No input handshake abstraction (exposes s_data_tvalid) and no rate propagation.
  Stage2_design : xbsIndex_r4/FDATool  block_type=fdatool
      settings: infoedit=FDATool
  Stage3_ch1-6 : xbsIndex_r4/FIR Compiler 7.2   coefficientvector=[-0.000008845311553949415216829832431244, -0.000027087054775247854738941949426234, -0.000055417714159712840797482324983747, -0.000087094432371299818095890243885293, -0.000105866390596641367599466121429685, -0.000085534137319013593420830021685219, 0.000006652205735310386510101068879841, 0.000201832685709543116926029115987262, 0.000516931678413450079213886656503973, 0.000939578230429354249557405420745226, 0.001414209115577612840483623379839173, 0.001834207533272972897100960842919903, 0.002045113408640639000857230911378792, 0.001862736203256826986868199824698422, 0.001107332948268861588445033383720783, -0.000348797711541245928149046484634254, -0.002527195112959597714241688493075344, -0.005293148036467960719508862865723131, -0.008322219080479574884745552765252796, -0.011095463689900950457478678856659826, -0.012931990944205273841305370297050103, -0.013061380366196617339169527838294015, -0.010730572542391882129297897563446895, -0.005331698470063657435691339969707769, 0.003469303386075768547147646359007922, 0.015626826872897403575279895449057221, 0.030655046242238678799729711954569211, 0.047629532261663394543393934554842417, 0.065258203667261274749655797222658293, 0.082016728321515186550527687359135597, 0.096331361203920634617148266443109605, 0.106782470317684924365764231879438739, 0.112296764341074842286083423914533341, 0.112296764341074842286083423914533341, 0.106782470317684924365764231879438739, 0.096331361203920634617148266443109605, 0.082016728321515186550527687359135597, 0.065258203667261274749655797222658293, 0.047629532261663394543393934554842417, 0.030655046242238678799729711954569211, 0.015626826872897403575279895449057221, 0.003469303386075768547147646359007922, -0.005331698470063657435691339969707769, -0.010730572542391882129297897563446895, -0.013061380366196617339169527838294015, -0.012931990944205273841305370297050103, -0.011095463689900950457478678856659826, -0.008322219080479574884745552765252796, -0.005293148036467960719508862865723131, -0.002527195112959597714241688493075344, -0.000348797711541245928149046484634254, 0.001107332948268861588445033383720783, 0.001862736203256826986868199824698422, 0.002045113408640639000857230911378792, 0.001834207533272972897100960842919903, 0.001414209115577612840483623379839173, 0.000939578230429354249557405420745226, 0.000516931678413450079213886656503973, 0.000201832685709543116926029115987262, 0.000006652205735310386510101068879841, -0.000085534137319013593420830021685219, -0.000105866390596641367599466121429685, -0.000087094432371299818095890243885293, -0.000055417714159712840797482324983747, -0.000027087054775247854738941949426234, -0.000008845311553949415216829832431244]  coefficient_sets=1  coefficient_reload=off  filter_type=Decimation  rate_change_type=Integer  interpolation_rate=1  decimation_rate=5  zero_pack_factor=1  channel_sequence=Basic  number_channels=1  pattern_list='P4-0,P4-1,P4-2,P4-3,P4-4'  number_paths=12  ratespecification=Maximum_Possible  sampleperiod=1  hardwareoversamplingrate=1  coefficient_sign=Signed  quantization=Maximize_Dynamic_Range  coefficient_width=25  bestprecision=off  coefficient_fractional_bits=24  coefficient_structure=Inferred  output_rounding_mode=Symmetric_Rounding_to_Infinity  output_width=32  filter_architecture=Systolic_Multiply_Accumulate  optimization_goal=Area  optimization_list='None'  data_buffer_type=Automatic  coefficient_buffer_type=Automatic  input_buffer_type=Automatic  output_buffer_type=Automatic  preference_for_other_storage=Automatic  multi_column_support=Automatic  columnconfig='7'  inter_column_pipe_length=4  data_has_tlast=Not_Required  m_data_has_tready=off  s_data_has_fifo=off  s_data_has_tuser=Not_Required  m_data_has_tuser=Not_Required  s_config_sync_mode=On_Vector  s_config_method=Single  num_reload_slots=1  has_aclken=off  has_aresetn=off  infoeditControl=ARESETn must be asserted for a minimum of 2 cycles  reset_data_vector=on  trim_axipin_name=on  simulation_type=hybrid_sim  simulation_model=sysgen:xfirv7_2_cmodel  data_path_portlist={ 's_axis_data_tdata', 'm_axis_data_tdata' }  passband_min=0.0  passband_max=0.5  stopband_min=0.5  stopband_max=1.0  filter_selection=1  gui_behaviour='Sysgen_GUI'  data_sign=Signed  data_width=16  data_fractional_bits=0  data_tuser_width=1  wrapper_available=true  ip_wrap_arbitrary_binary_point=true  ip_name=FIR Compiler  ip_version=7.2  dsptool_ready=true  ipcore_usecache=true  ipcore_useipmodelcache=true  port_translation_map={ 'aclken' => 'en', 'aresetn' => 'rst' }  run_core_at_system_period=true  ipcore_xco_need_fpga_part=true  block_type=fir_compiler_v7_2
      settings: infoedit=Maximum Possible : Maximizes oversampling rate. Abstracted input handshake (no s_data_tvalid) and automatic rate propagation.<br>Hardware Oversampling Rate : Specifies oversampling rate relative to the input sample period. Abstracted input handshake (no s_data_tvalid) and automatic rate propagation.<br>Input/Output Sample Period : Specifies absolute oversampling rate. No input handshake abstraction (exposes s_data_tvalid) and no rate propagation.
  Stage3_ch7-10 : xbsIndex_r4/FIR Compiler 7.2   coefficientvector=[-0.000008845311553949415216829832431244, -0.000027087054775247854738941949426234, -0.000055417714159712840797482324983747, -0.000087094432371299818095890243885293, -0.000105866390596641367599466121429685, -0.000085534137319013593420830021685219, 0.000006652205735310386510101068879841, 0.000201832685709543116926029115987262, 0.000516931678413450079213886656503973, 0.000939578230429354249557405420745226, 0.001414209115577612840483623379839173, 0.001834207533272972897100960842919903, 0.002045113408640639000857230911378792, 0.001862736203256826986868199824698422, 0.001107332948268861588445033383720783, -0.000348797711541245928149046484634254, -0.002527195112959597714241688493075344, -0.005293148036467960719508862865723131, -0.008322219080479574884745552765252796, -0.011095463689900950457478678856659826, -0.012931990944205273841305370297050103, -0.013061380366196617339169527838294015, -0.010730572542391882129297897563446895, -0.005331698470063657435691339969707769, 0.003469303386075768547147646359007922, 0.015626826872897403575279895449057221, 0.030655046242238678799729711954569211, 0.047629532261663394543393934554842417, 0.065258203667261274749655797222658293, 0.082016728321515186550527687359135597, 0.096331361203920634617148266443109605, 0.106782470317684924365764231879438739, 0.112296764341074842286083423914533341, 0.112296764341074842286083423914533341, 0.106782470317684924365764231879438739, 0.096331361203920634617148266443109605, 0.082016728321515186550527687359135597, 0.065258203667261274749655797222658293, 0.047629532261663394543393934554842417, 0.030655046242238678799729711954569211, 0.015626826872897403575279895449057221, 0.003469303386075768547147646359007922, -0.005331698470063657435691339969707769, -0.010730572542391882129297897563446895, -0.013061380366196617339169527838294015, -0.012931990944205273841305370297050103, -0.011095463689900950457478678856659826, -0.008322219080479574884745552765252796, -0.005293148036467960719508862865723131, -0.002527195112959597714241688493075344, -0.000348797711541245928149046484634254, 0.001107332948268861588445033383720783, 0.001862736203256826986868199824698422, 0.002045113408640639000857230911378792, 0.001834207533272972897100960842919903, 0.001414209115577612840483623379839173, 0.000939578230429354249557405420745226, 0.000516931678413450079213886656503973, 0.000201832685709543116926029115987262, 0.000006652205735310386510101068879841, -0.000085534137319013593420830021685219, -0.000105866390596641367599466121429685, -0.000087094432371299818095890243885293, -0.000055417714159712840797482324983747, -0.000027087054775247854738941949426234, -0.000008845311553949415216829832431244]  coefficient_sets=1  coefficient_reload=off  filter_type=Decimation  rate_change_type=Integer  interpolation_rate=1  decimation_rate=5  zero_pack_factor=1  channel_sequence=Basic  number_channels=1  pattern_list='P4-0,P4-1,P4-2,P4-3,P4-4'  number_paths=8  ratespecification=Maximum_Possible  sampleperiod=1  hardwareoversamplingrate=1  coefficient_sign=Signed  quantization=Maximize_Dynamic_Range  coefficient_width=25  bestprecision=off  coefficient_fractional_bits=24  coefficient_structure=Inferred  output_rounding_mode=Symmetric_Rounding_to_Infinity  output_width=32  filter_architecture=Systolic_Multiply_Accumulate  optimization_goal=Area  optimization_list='None'  data_buffer_type=Automatic  coefficient_buffer_type=Automatic  input_buffer_type=Automatic  output_buffer_type=Automatic  preference_for_other_storage=Automatic  multi_column_support=Automatic  columnconfig='7'  inter_column_pipe_length=4  data_has_tlast=Not_Required  m_data_has_tready=off  s_data_has_fifo=off  s_data_has_tuser=Not_Required  m_data_has_tuser=Not_Required  s_config_sync_mode=On_Vector  s_config_method=Single  num_reload_slots=1  has_aclken=off  has_aresetn=off  infoeditControl=ARESETn must be asserted for a minimum of 2 cycles  reset_data_vector=on  trim_axipin_name=on  simulation_type=hybrid_sim  simulation_model=sysgen:xfirv7_2_cmodel  data_path_portlist={ 's_axis_data_tdata', 'm_axis_data_tdata' }  passband_min=0.0  passband_max=0.5  stopband_min=0.5  stopband_max=1.0  filter_selection=1  gui_behaviour='Sysgen_GUI'  data_sign=Signed  data_width=16  data_fractional_bits=0  data_tuser_width=1  wrapper_available=true  ip_wrap_arbitrary_binary_point=true  ip_name=FIR Compiler  ip_version=7.2  dsptool_ready=true  ipcore_usecache=true  ipcore_useipmodelcache=true  port_translation_map={ 'aclken' => 'en', 'aresetn' => 'rst' }  run_core_at_system_period=true  ipcore_xco_need_fpga_part=true  block_type=fir_compiler_v7_2
      settings: infoedit=Maximum Possible : Maximizes oversampling rate. Abstracted input handshake (no s_data_tvalid) and automatic rate propagation.<br>Hardware Oversampling Rate : Specifies oversampling rate relative to the input sample period. Abstracted input handshake (no s_data_tvalid) and automatic rate propagation.<br>Input/Output Sample Period : Specifies absolute oversampling rate. No input handshake abstraction (exposes s_data_tvalid) and no rate propagation.
  Stage3_design : xbsIndex_r4/FDATool  block_type=fdatool
      settings: infoedit=FDATool
  Stage4_ch1-6 : xbsIndex_r4/FIR Compiler 7.2   coefficientvector=[-0.000020100983725471430218524615529673, -0.000039300117033273202307198934679632, -0.000044010763301423614149692625785448, -0.000010573356963638086978077290645217, 0.000074844700889607274681830650919778, 0.000198041523378862855710169643685958, 0.000306512114498588394539274615269164, 0.000318597772408086112646413701199321, 0.000156869734231666072216473950540205, -0.000202162914157001514419212395701208, -0.000683547331713031886338272080649858, -0.001102945587947771772380223254117481, -0.001211070052905736287376936566317908, -0.000793931134816088196308470070761131, 0.000200624156115792489415289301390998, 0.001565123661435297020005918966489844, 0.002824583917525473868853636005837870, 0.003356711444245746162051702299322641, 0.002628502921894513427725215137797931, 0.000477083709614566813580344151191070, -0.002682195806059435843476945748875550, -0.005840531950413944961564283175903256, -0.007641674729585433943623851149595793, -0.006859866127731274396128746673184650, -0.002969150702903962726897368895606632, 0.003415141575091562489013830017370310, 0.010445687700825321761466391023986943, 0.015436262163650016354665694962022826, 0.015705653736096725214821390181896276, 0.009650632996108471015062058029343461, -0.002312739010546308471988341537439737, -0.017324277028273164097393888027909270, -0.030436169465888680829568357921743881, -0.035775248316263157100092229256915743, -0.028248756647164051380993754492010339, -0.005299969304667222734506193404513396, 0.031863512847745856237935413446393795, 0.078035050068266526013260886429634410, 0.124949995715424463926801479374262271, 0.163214051552529909594468904288078192, 0.184697636593445402297675173031166195, 0.184697636593445402297675173031166195, 0.163214051552529909594468904288078192, 0.124949995715424463926801479374262271, 0.078035050068266526013260886429634410, 0.031863512847745856237935413446393795, -0.005299969304667222734506193404513396, -0.028248756647164051380993754492010339, -0.035775248316263157100092229256915743, -0.030436169465888680829568357921743881, -0.017324277028273164097393888027909270, -0.002312739010546308471988341537439737, 0.009650632996108471015062058029343461, 0.015705653736096725214821390181896276, 0.015436262163650016354665694962022826, 0.010445687700825321761466391023986943, 0.003415141575091562489013830017370310, -0.002969150702903962726897368895606632, -0.006859866127731274396128746673184650, -0.007641674729585433943623851149595793, -0.005840531950413944961564283175903256, -0.002682195806059435843476945748875550, 0.000477083709614566813580344151191070, 0.002628502921894513427725215137797931, 0.003356711444245746162051702299322641, 0.002824583917525473868853636005837870, 0.001565123661435297020005918966489844, 0.000200624156115792489415289301390998, -0.000793931134816088196308470070761131, -0.001211070052905736287376936566317908, -0.001102945587947771772380223254117481, -0.000683547331713031886338272080649858, -0.000202162914157001514419212395701208, 0.000156869734231666072216473950540205, 0.000318597772408086112646413701199321, 0.000306512114498588394539274615269164, 0.000198041523378862855710169643685958, 0.000074844700889607274681830650919778, -0.000010573356963638086978077290645217, -0.000044010763301423614149692625785448, -0.000039300117033273202307198934679632, -0.000020100983725471430218524615529673]  coefficient_sets=1  coefficient_reload=off  filter_type=Decimation  rate_change_type=Integer  interpolation_rate=1  decimation_rate=4  zero_pack_factor=1  channel_sequence=Basic  number_channels=1  pattern_list='P4-0,P4-1,P4-2,P4-3,P4-4'  number_paths=12  ratespecification=Maximum_Possible  sampleperiod=1  hardwareoversamplingrate=1  coefficient_sign=Signed  quantization=Maximize_Dynamic_Range  coefficient_width=25  bestprecision=off  coefficient_fractional_bits=24  coefficient_structure=Inferred  output_rounding_mode=Symmetric_Rounding_to_Infinity  output_width=32  filter_architecture=Systolic_Multiply_Accumulate  optimization_goal=Area  optimization_list='None'  data_buffer_type=Automatic  coefficient_buffer_type=Automatic  input_buffer_type=Automatic  output_buffer_type=Automatic  preference_for_other_storage=Automatic  multi_column_support=Automatic  columnconfig='11'  inter_column_pipe_length=4  data_has_tlast=Not_Required  m_data_has_tready=off  s_data_has_fifo=off  s_data_has_tuser=Not_Required  m_data_has_tuser=Not_Required  s_config_sync_mode=On_Vector  s_config_method=Single  num_reload_slots=1  has_aclken=off  has_aresetn=off  infoeditControl=ARESETn must be asserted for a minimum of 2 cycles  reset_data_vector=on  trim_axipin_name=on  simulation_type=hybrid_sim  simulation_model=sysgen:xfirv7_2_cmodel  data_path_portlist={ 's_axis_data_tdata', 'm_axis_data_tdata' }  passband_min=0.0  passband_max=0.5  stopband_min=0.5  stopband_max=1.0  filter_selection=1  gui_behaviour='Sysgen_GUI'  data_sign=Signed  data_width=16  data_fractional_bits=0  data_tuser_width=1  wrapper_available=true  ip_wrap_arbitrary_binary_point=true  ip_name=FIR Compiler  ip_version=7.2  dsptool_ready=true  ipcore_usecache=true  ipcore_useipmodelcache=true  port_translation_map={ 'aclken' => 'en', 'aresetn' => 'rst' }  run_core_at_system_period=true  ipcore_xco_need_fpga_part=true  block_type=fir_compiler_v7_2
      settings: infoedit=Maximum Possible : Maximizes oversampling rate. Abstracted input handshake (no s_data_tvalid) and automatic rate propagation.<br>Hardware Oversampling Rate : Specifies oversampling rate relative to the input sample period. Abstracted input handshake (no s_data_tvalid) and automatic rate propagation.<br>Input/Output Sample Period : Specifies absolute oversampling rate. No input handshake abstraction (exposes s_data_tvalid) and no rate propagation.
  Stage4_ch7-10 : xbsIndex_r4/FIR Compiler 7.2   coefficientvector=[-0.000020100983725471430218524615529673, -0.000039300117033273202307198934679632, -0.000044010763301423614149692625785448, -0.000010573356963638086978077290645217, 0.000074844700889607274681830650919778, 0.000198041523378862855710169643685958, 0.000306512114498588394539274615269164, 0.000318597772408086112646413701199321, 0.000156869734231666072216473950540205, -0.000202162914157001514419212395701208, -0.000683547331713031886338272080649858, -0.001102945587947771772380223254117481, -0.001211070052905736287376936566317908, -0.000793931134816088196308470070761131, 0.000200624156115792489415289301390998, 0.001565123661435297020005918966489844, 0.002824583917525473868853636005837870, 0.003356711444245746162051702299322641, 0.002628502921894513427725215137797931, 0.000477083709614566813580344151191070, -0.002682195806059435843476945748875550, -0.005840531950413944961564283175903256, -0.007641674729585433943623851149595793, -0.006859866127731274396128746673184650, -0.002969150702903962726897368895606632, 0.003415141575091562489013830017370310, 0.010445687700825321761466391023986943, 0.015436262163650016354665694962022826, 0.015705653736096725214821390181896276, 0.009650632996108471015062058029343461, -0.002312739010546308471988341537439737, -0.017324277028273164097393888027909270, -0.030436169465888680829568357921743881, -0.035775248316263157100092229256915743, -0.028248756647164051380993754492010339, -0.005299969304667222734506193404513396, 0.031863512847745856237935413446393795, 0.078035050068266526013260886429634410, 0.124949995715424463926801479374262271, 0.163214051552529909594468904288078192, 0.184697636593445402297675173031166195, 0.184697636593445402297675173031166195, 0.163214051552529909594468904288078192, 0.124949995715424463926801479374262271, 0.078035050068266526013260886429634410, 0.031863512847745856237935413446393795, -0.005299969304667222734506193404513396, -0.028248756647164051380993754492010339, -0.035775248316263157100092229256915743, -0.030436169465888680829568357921743881, -0.017324277028273164097393888027909270, -0.002312739010546308471988341537439737, 0.009650632996108471015062058029343461, 0.015705653736096725214821390181896276, 0.015436262163650016354665694962022826, 0.010445687700825321761466391023986943, 0.003415141575091562489013830017370310, -0.002969150702903962726897368895606632, -0.006859866127731274396128746673184650, -0.007641674729585433943623851149595793, -0.005840531950413944961564283175903256, -0.002682195806059435843476945748875550, 0.000477083709614566813580344151191070, 0.002628502921894513427725215137797931, 0.003356711444245746162051702299322641, 0.002824583917525473868853636005837870, 0.001565123661435297020005918966489844, 0.000200624156115792489415289301390998, -0.000793931134816088196308470070761131, -0.001211070052905736287376936566317908, -0.001102945587947771772380223254117481, -0.000683547331713031886338272080649858, -0.000202162914157001514419212395701208, 0.000156869734231666072216473950540205, 0.000318597772408086112646413701199321, 0.000306512114498588394539274615269164, 0.000198041523378862855710169643685958, 0.000074844700889607274681830650919778, -0.000010573356963638086978077290645217, -0.000044010763301423614149692625785448, -0.000039300117033273202307198934679632, -0.000020100983725471430218524615529673]  coefficient_sets=1  coefficient_reload=off  filter_type=Decimation  rate_change_type=Integer  interpolation_rate=1  decimation_rate=4  zero_pack_factor=1  channel_sequence=Basic  number_channels=1  pattern_list='P4-0,P4-1,P4-2,P4-3,P4-4'  number_paths=8  ratespecification=Maximum_Possible  sampleperiod=1  hardwareoversamplingrate=1  coefficient_sign=Signed  quantization=Maximize_Dynamic_Range  coefficient_width=25  bestprecision=off  coefficient_fractional_bits=24  coefficient_structure=Inferred  output_rounding_mode=Symmetric_Rounding_to_Infinity  output_width=32  filter_architecture=Systolic_Multiply_Accumulate  optimization_goal=Area  optimization_list='None'  data_buffer_type=Automatic  coefficient_buffer_type=Automatic  input_buffer_type=Automatic  output_buffer_type=Automatic  preference_for_other_storage=Automatic  multi_column_support=Automatic  columnconfig='11'  inter_column_pipe_length=4  data_has_tlast=Not_Required  m_data_has_tready=off  s_data_has_fifo=off  s_data_has_tuser=Not_Required  m_data_has_tuser=Not_Required  s_config_sync_mode=On_Vector  s_config_method=Single  num_reload_slots=1  has_aclken=off  has_aresetn=off  infoeditControl=ARESETn must be asserted for a minimum of 2 cycles  reset_data_vector=on  trim_axipin_name=on  simulation_type=hybrid_sim  simulation_model=sysgen:xfirv7_2_cmodel  data_path_portlist={ 's_axis_data_tdata', 'm_axis_data_tdata' }  passband_min=0.0  passband_max=0.5  stopband_min=0.5  stopband_max=1.0  filter_selection=1  gui_behaviour='Sysgen_GUI'  data_sign=Signed  data_width=16  data_fractional_bits=0  data_tuser_width=1  wrapper_available=true  ip_wrap_arbitrary_binary_point=true  ip_name=FIR Compiler  ip_version=7.2  dsptool_ready=true  ipcore_usecache=true  ipcore_useipmodelcache=true  port_translation_map={ 'aclken' => 'en', 'aresetn' => 'rst' }  run_core_at_system_period=true  ipcore_xco_need_fpga_part=true  block_type=fir_compiler_v7_2
      settings: infoedit=Maximum Possible : Maximizes oversampling rate. Abstracted input handshake (no s_data_tvalid) and automatic rate propagation.<br>Hardware Oversampling Rate : Specifies oversampling rate relative to the input sample period. Abstracted input handshake (no s_data_tvalid) and automatic rate propagation.<br>Input/Output Sample Period : Specifies absolute oversampling rate. No input handshake abstraction (exposes s_data_tvalid) and no rate propagation.
  Stage4_design : xbsIndex_r4/FDATool  block_type=fdatool
      settings: infoedit=FDATool
  Stage5_ch1-6 : xbsIndex_r4/FIR Compiler 7.2   coefficientvector=[0.000007330468028988360409178154375453, 0.000001061375341940230003086559178171, -0.000008302375967268891537452664419749, -0.000001310478879802316095324644928954, 0.000009334193535475371279784909117616, 0.000001595555133339845714054625568090, -0.000010427587541815879423282714677512, -0.000001919438945047465104479320757713, 0.000011584197613561845959006049722184, 0.000002285084523029715418358841574897, -0.000012805632251774457517397992623031, -0.000002695566914179534686712286228882, 0.000014093464790261419147679791685767, 0.000003154083380998819414396368635000, -0.000015449229261449387806638330888908, -0.000003663954678804840236111583021139, 0.000016874416172015358790633662855462, 0.000004228626230212040421302215065235, -0.000018370468191260861626646488931058, -0.000004851669193878087733536388914679, 0.000019938775755349383978073593559621, 0.000005536781424697596465519470326777, -0.000021580672590681486920898696224568, -0.000006287788322803664813141072409408, 0.000023297431159783956068761931468280, 0.000007108643568852213902461122108089, -0.000025090258033248307557123643607432, -0.000008003429743300613158677424274767, 0.000026960289191331901704129156427391, 0.000008976358827600000001262041393612, -0.000028908585258986339551695934901864, -0.000010031772585349056563599513813844, 0.000030936126678142249592576296102208, 0.000011174142821737787393079378850391, -0.000033043808821202832223633272246132, -0.000012408071519848629145755906921788, 0.000035232437049774135626439147683797, 0.000013738290852522787560251876781691, -0.000037502721722719207109869588023798, -0.000015169663068825736917640337186874, 0.000039855273157729979936324954392645, 0.000016707180254418878593376460162112, -0.000042290596550637315218304501662771, -0.000018355963965275345564512679552571, 0.000044809086856713625150825525134123, 0.000020121264734617554917252973956109, -0.000047411023638316602429355894887663, -0.000022008461453128109601993026012145, 0.000050096565883171975566527656109627, 0.000024023060622783862184601022526919, -0.000052865746797662212512914498008242, -0.000026170695485037191133515649399399, 0.000055718468579447654246122184629186, 0.000028457125024291475865823378144092, -0.000058654497173782697806102698345753, -0.000030888232848017749450093144547579, 0.000061673457017769010434123100328207, 0.000033470025945079102849388091867055, -0.000064774825776865900344402005028854, -0.000036208633324377922631329834723956, 0.000067957929077834536486270311517188, 0.000039110304536019479323006448057142, -0.000071221935242202165220783138810389, -0.000042181408077743920502066660160878, 0.000074565850024349588677508027245721, 0.000045428429689773650132934151857355, -0.000077988511358123406309178493600597, -0.000048857970541388734972768070896620, 0.000081488584115725477244503160978439, 0.000052476745313136440647828334649105, -0.000085064554882625657470339441967865, -0.000056291580179014084558703628902165, 0.000088714726751960360558862950242087, 0.000060309410693130180837560200268754, -0.000092437214141668803068195570116216, -0.000064537279586008122040340084790699, 0.000096229937637586337442416328791239, 0.000068982334476163262543084442324214, -0.000100090618865334546978493324154158, -0.000073651825502754535786482936732255, 0.000104016775393573785986160717964565, 0.000078553102885840395911559719266392, -0.000108005715671114676168160229074999, -0.000083693614421272432028417465055269, 0.000112054533999904904211127043556217, 0.000089080902917440258747400205763256, -0.000116160105545547073487358535892610, -0.000094722603581880092881405130977867, 0.000120319081386942064687377296205994, 0.000100626441366321361437809189798286, -0.000124527883605910020528226289648898, -0.000106800228278874272396133104923166, 0.000128782700417471961248580547554354, 0.000113251860673152353071319042854270, -0.000133079481341031409177833033652404, -0.000119989316524287350129891749350719, 0.000137413932412058824913264620803943, 0.000127020652702632054920767190608899, ...(+24783 chars)]  coefficient_sets=1  coefficient_reload=off  filter_type=Decimation  rate_change_type=Integer  interpolation_rate=1  decimation_rate=2  zero_pack_factor=1  channel_sequence=Basic  number_channels=1  pattern_list='P4-0,P4-1,P4-2,P4-3,P4-4'  number_paths=12  ratespecification=Maximum_Possible  sampleperiod=1  hardwareoversamplingrate=1  coefficient_sign=Signed  quantization=Maximize_Dynamic_Range  coefficient_width=25  bestprecision=off  coefficient_fractional_bits=24  coefficient_structure=Inferred  output_rounding_mode=Symmetric_Rounding_to_Infinity  output_width=32  filter_architecture=Systolic_Multiply_Accumulate  optimization_goal=Area  optimization_list='None'  data_buffer_type=Automatic  coefficient_buffer_type=Automatic  input_buffer_type=Automatic  output_buffer_type=Automatic  preference_for_other_storage=Automatic  multi_column_support=Automatic  columnconfig='178'  inter_column_pipe_length=4  data_has_tlast=Not_Required  m_data_has_tready=off  s_data_has_fifo=off  s_data_has_tuser=Not_Required  m_data_has_tuser=Not_Required  s_config_sync_mode=On_Vector  s_config_method=Single  num_reload_slots=1  has_aclken=off  has_aresetn=off  infoeditControl=ARESETn must be asserted for a minimum of 2 cycles  reset_data_vector=on  trim_axipin_name=on  simulation_type=hybrid_sim  simulation_model=sysgen:xfirv7_2_cmodel  data_path_portlist={ 's_axis_data_tdata', 'm_axis_data_tdata' }  passband_min=0.0  passband_max=0.5  stopband_min=0.5  stopband_max=1.0  filter_selection=1  gui_behaviour='Sysgen_GUI'  data_sign=Signed  data_width=16  data_fractional_bits=0  data_tuser_width=1  wrapper_available=true  ip_wrap_arbitrary_binary_point=true  ip_name=FIR Compiler  ip_version=7.2  dsptool_ready=true  ipcore_usecache=true  ipcore_useipmodelcache=true  port_translation_map={ 'aclken' => 'en', 'aresetn' => 'rst' }  run_core_at_system_period=true  ipcore_xco_need_fpga_part=true  block_type=fir_compiler_v7_2
      settings: infoedit=Maximum Possible : Maximizes oversampling rate. Abstracted input handshake (no s_data_tvalid) and automatic rate propagation.<br>Hardware Oversampling Rate : Specifies oversampling rate relative to the input sample period. Abstracted input handshake (no s_data_tvalid) and automatic rate propagation.<br>Input/Output Sample Period : Specifies absolute oversampling rate. No input handshake abstraction (exposes s_data_tvalid) and no rate propagation.
  Stage5_ch7-10 : xbsIndex_r4/FIR Compiler 7.2   coefficientvector=[0.000007330468028988360409178154375453, 0.000001061375341940230003086559178171, -0.000008302375967268891537452664419749, -0.000001310478879802316095324644928954, 0.000009334193535475371279784909117616, 0.000001595555133339845714054625568090, -0.000010427587541815879423282714677512, -0.000001919438945047465104479320757713, 0.000011584197613561845959006049722184, 0.000002285084523029715418358841574897, -0.000012805632251774457517397992623031, -0.000002695566914179534686712286228882, 0.000014093464790261419147679791685767, 0.000003154083380998819414396368635000, -0.000015449229261449387806638330888908, -0.000003663954678804840236111583021139, 0.000016874416172015358790633662855462, 0.000004228626230212040421302215065235, -0.000018370468191260861626646488931058, -0.000004851669193878087733536388914679, 0.000019938775755349383978073593559621, 0.000005536781424697596465519470326777, -0.000021580672590681486920898696224568, -0.000006287788322803664813141072409408, 0.000023297431159783956068761931468280, 0.000007108643568852213902461122108089, -0.000025090258033248307557123643607432, -0.000008003429743300613158677424274767, 0.000026960289191331901704129156427391, 0.000008976358827600000001262041393612, -0.000028908585258986339551695934901864, -0.000010031772585349056563599513813844, 0.000030936126678142249592576296102208, 0.000011174142821737787393079378850391, -0.000033043808821202832223633272246132, -0.000012408071519848629145755906921788, 0.000035232437049774135626439147683797, 0.000013738290852522787560251876781691, -0.000037502721722719207109869588023798, -0.000015169663068825736917640337186874, 0.000039855273157729979936324954392645, 0.000016707180254418878593376460162112, -0.000042290596550637315218304501662771, -0.000018355963965275345564512679552571, 0.000044809086856713625150825525134123, 0.000020121264734617554917252973956109, -0.000047411023638316602429355894887663, -0.000022008461453128109601993026012145, 0.000050096565883171975566527656109627, 0.000024023060622783862184601022526919, -0.000052865746797662212512914498008242, -0.000026170695485037191133515649399399, 0.000055718468579447654246122184629186, 0.000028457125024291475865823378144092, -0.000058654497173782697806102698345753, -0.000030888232848017749450093144547579, 0.000061673457017769010434123100328207, 0.000033470025945079102849388091867055, -0.000064774825776865900344402005028854, -0.000036208633324377922631329834723956, 0.000067957929077834536486270311517188, 0.000039110304536019479323006448057142, -0.000071221935242202165220783138810389, -0.000042181408077743920502066660160878, 0.000074565850024349588677508027245721, 0.000045428429689773650132934151857355, -0.000077988511358123406309178493600597, -0.000048857970541388734972768070896620, 0.000081488584115725477244503160978439, 0.000052476745313136440647828334649105, -0.000085064554882625657470339441967865, -0.000056291580179014084558703628902165, 0.000088714726751960360558862950242087, 0.000060309410693130180837560200268754, -0.000092437214141668803068195570116216, -0.000064537279586008122040340084790699, 0.000096229937637586337442416328791239, 0.000068982334476163262543084442324214, -0.000100090618865334546978493324154158, -0.000073651825502754535786482936732255, 0.000104016775393573785986160717964565, 0.000078553102885840395911559719266392, -0.000108005715671114676168160229074999, -0.000083693614421272432028417465055269, 0.000112054533999904904211127043556217, 0.000089080902917440258747400205763256, -0.000116160105545547073487358535892610, -0.000094722603581880092881405130977867, 0.000120319081386942064687377296205994, 0.000100626441366321361437809189798286, -0.000124527883605910020528226289648898, -0.000106800228278874272396133104923166, 0.000128782700417471961248580547554354, 0.000113251860673152353071319042854270, -0.000133079481341031409177833033652404, -0.000119989316524287350129891749350719, 0.000137413932412058824913264620803943, 0.000127020652702632054920767190608899, ...(+24783 chars)]  coefficient_sets=1  coefficient_reload=off  filter_type=Decimation  rate_change_type=Integer  interpolation_rate=1  decimation_rate=2  zero_pack_factor=1  channel_sequence=Basic  number_channels=1  pattern_list='P4-0,P4-1,P4-2,P4-3,P4-4'  number_paths=8  ratespecification=Maximum_Possible  sampleperiod=1  hardwareoversamplingrate=1  coefficient_sign=Signed  quantization=Maximize_Dynamic_Range  coefficient_width=25  bestprecision=off  coefficient_fractional_bits=24  coefficient_structure=Inferred  output_rounding_mode=Symmetric_Rounding_to_Infinity  output_width=32  filter_architecture=Systolic_Multiply_Accumulate  optimization_goal=Area  optimization_list='None'  data_buffer_type=Automatic  coefficient_buffer_type=Automatic  input_buffer_type=Automatic  output_buffer_type=Automatic  preference_for_other_storage=Automatic  multi_column_support=Automatic  columnconfig='50,24'  inter_column_pipe_length=4  data_has_tlast=Not_Required  m_data_has_tready=off  s_data_has_fifo=off  s_data_has_tuser=Not_Required  m_data_has_tuser=Not_Required  s_config_sync_mode=On_Vector  s_config_method=Single  num_reload_slots=1  has_aclken=off  has_aresetn=off  infoeditControl=ARESETn must be asserted for a minimum of 2 cycles  reset_data_vector=on  trim_axipin_name=on  simulation_type=hybrid_sim  simulation_model=sysgen:xfirv7_2_cmodel  data_path_portlist={ 's_axis_data_tdata', 'm_axis_data_tdata' }  passband_min=0.0  passband_max=0.5  stopband_min=0.5  stopband_max=1.0  filter_selection=1  gui_behaviour='Sysgen_GUI'  data_sign=Signed  data_width=16  data_fractional_bits=0  data_tuser_width=1  wrapper_available=true  ip_wrap_arbitrary_binary_point=true  ip_name=FIR Compiler  ip_version=7.2  dsptool_ready=true  ipcore_usecache=true  ipcore_useipmodelcache=true  port_translation_map={ 'aclken' => 'en', 'aresetn' => 'rst' }  run_core_at_system_period=true  ipcore_xco_need_fpga_part=true  block_type=fir_compiler_v7_2
      settings: infoedit=Maximum Possible : Maximizes oversampling rate. Abstracted input handshake (no s_data_tvalid) and automatic rate propagation.<br>Hardware Oversampling Rate : Specifies oversampling rate relative to the input sample period. Abstracted input handshake (no s_data_tvalid) and automatic rate propagation.<br>Input/Output Sample Period : Specifies absolute oversampling rate. No input handshake abstraction (exposes s_data_tvalid) and no rate propagation.
  Stage5_design : xbsIndex_r4/FDATool  block_type=fdatool
      settings: infoedit=FDATool
  Terminator{1..38,40,43,45..46,48..49} (44 alike) : Terminator
  dest_ip : Subsystem  Tag=xps:sw_reg  AncestorBlock=xps_library/Memory/software_register  mask(swreg){io_dir=From Processor, io_delay=0, init_val=0, sample_period=1, names=reg, bitwidths=32, bin_pts=0, arith_types=0, sim_port=on, show_format=on}
      mask prompts: io_dir "I/O direction"; io_delay "I/O delay"; init_val "Initial Value"; sample_period "Sample period"; names "Bitfield names [msb...lsb]"; bitwidths "Bitfield widths"; bin_pts "Bitfield binary pts"; arith_types "Bitfield types, ufix=0, fix=1, bool=2"; sim_port "Provide sim input/output?"; show_format "Print format string?"
      mask help: A 32-bit software-accessible register. Can be divided into bitfields of varying widths and types using the fields in the block mask.
      mask init:
      | swreg_init(gcb)
      settings: AttributesFormatString=1input:uf32.0 = 32 bits
      mask TypeOptions io_dir: To Processor | From Processor
      mask Callback io_dir:
      | mask_enables = get_param(gcb, 'MaskEnables');
      | mask_names = get_param(gcb, 'MaskNames');
      | if strcmp(get_param(gcb, 'io_dir'), 'To Processor'),
      |     mask_enables{ismember(mask_names, 'sample_period')} = 'off';
      | else
      |     mask_enables{ismember(mask_names, 'sample_period')} = 'on';
      | end
      | set_param(gcb, 'MaskEnables', mask_enables);
      mask DialogControl ParameterTabVar0 Prompt: Setup
  dest_port : Subsystem  Tag=xps:sw_reg  AncestorBlock=xps_library/Memory/software_register  mask(swreg){io_dir=From Processor, io_delay=0, init_val=0, sample_period=1, names=reg, bitwidths=16, bin_pts=0, arith_types=0, sim_port=on, show_format=on}
      mask prompts: io_dir "I/O direction"; io_delay "I/O delay"; init_val "Initial Value"; sample_period "Sample period"; names "Bitfield names [msb...lsb]"; bitwidths "Bitfield widths"; bin_pts "Bitfield binary pts"; arith_types "Bitfield types, ufix=0, fix=1, bool=2"; sim_port "Provide sim input/output?"; show_format "Print format string?"
      mask help: A 32-bit software-accessible register. Can be divided into bitfields of varying widths and types using the fields in the block mask.
      mask init:
      | swreg_init(gcb)
      settings: AttributesFormatString=1input:uf16.0 = 16 bits
      mask TypeOptions io_dir: To Processor | From Processor
      mask Callback io_dir:
      | mask_enables = get_param(gcb, 'MaskEnables');
      | mask_names = get_param(gcb, 'MaskNames');
      | if strcmp(get_param(gcb, 'io_dir'), 'To Processor'),
      |     mask_enables{ismember(mask_names, 'sample_period')} = 'off';
      | else
      |     mask_enables{ismember(mask_names, 'sample_period')} = 'on';
      | end
      | set_param(gcb, 'MaskEnables', mask_enables);
      mask DialogControl ParameterTabVar0 Prompt: Setup
  edge_detect1 : Subsystem  AncestorBlock=casper_library_misc/edge_detect  mask(edge_detect){edge=Rising, polarity=Active High, x_in=[0 0.08 0.08 0.16 0.16 0.24 0.24 0.32 0.32 0.4], y_in=[-1 -1  1  1  1  1  1  1  1  1], x_out=[0.6 0.68 0.68 0.76 0.76 0.84 0.84 0.92 0.92 1], y_out=[-1 -1  1  1 -1 -1 -1 -1 -1 -1]}
      mask prompts: edge "Edge Type"; polarity "Output Polarity"; x_in "Input X Positions"; y_in "Input Y Positions"; x_out "Output X Positions"; y_out "Output Y Positions"
      mask help: Output is active for one-cycle after each edge of the specified type (i.e. rising, falling or both).
      mask init:
      | edge_detect_init(gcb,...
      |     'edge',edge,...
      |     'polarity',polarity,...
      |     'x_in',x_in,...
      |     'x_out',x_out,...
      |     'y_in',y_in,...
      |     'y_out',y_out);
      | 
      | x_in_num=str2num(getfield(getfield(get_param(gcb,'UserData'),'parameters'),'x_in'));
      | x_out_num=str2num(getfield(getfield(get_param(gcb,'UserData'),'parameters'),'x_out'));
      | y_in_num=str2num(getfield(getfield(get_param(gcb,'UserData'),'parameters'),'y_in'));
      | y_out_num=str2num(getfield(getfield(get_param(gcb,'UserData'),'parameters'),'y_out'));
      settings: AttributesFormatString=|
      | rising edges
      | active high
      mask Help: Output is active for one-cycle after each edge of the specified type (i.e. rising, falling, or both).  Latency is zero.
      mask TypeOptions edge: Rising | Falling | Both
      mask TypeOptions polarity: Active High | Active Low
      mask Display:
      | plot(x_in_num,0.5+y_in_num*0.2);
      | plot(x_out_num,0.5+y_out_num*0.2);
  edge_detect2 : Subsystem  AncestorBlock=casper_library_misc/edge_detect  mask(edge_detect){edge=Rising, polarity=Active High, x_in=[0 0.08 0.08 0.16 0.16 0.24 0.24 0.32 0.32 0.4], y_in=[-1 -1  1  1  1  1  1  1  1  1], x_out=[0.6 0.68 0.68 0.76 0.76 0.84 0.84 0.92 0.92 1], y_out=[-1 -1  1  1 -1 -1 -1 -1 -1 -1]}
      mask prompts: edge "Edge Type"; polarity "Output Polarity"; x_in "Input X Positions"; y_in "Input Y Positions"; x_out "Output X Positions"; y_out "Output Y Positions"
      mask help: Output is active for one-cycle after each edge of the specified type (i.e. rising, falling or both).
      mask init: same as mdt_snap_10ch_daq/edge_detect1
      settings: AttributesFormatString=|
      | rising edges
      | active high
      mask Help: Output is active for one-cycle after each edge of the specified type (i.e. rising, falling, or both).  Latency is zero.
      mask TypeOptions edge: Rising | Falling | Both
      mask TypeOptions polarity: Active High | Active Low
      mask Display:
      | plot(x_in_num,0.5+y_in_num*0.2);
      | plot(x_out_num,0.5+y_out_num*0.2);
  edge_detect4 : Subsystem  AncestorBlock=casper_library_misc/edge_detect  mask(edge_detect){edge=Rising, polarity=Active High, x_in=[0 0.08 0.08 0.16 0.16 0.24 0.24 0.32 0.32 0.4], y_in=[-1 -1  1  1  1  1  1  1  1  1], x_out=[0.6 0.68 0.68 0.76 0.76 0.84 0.84 0.92 0.92 1], y_out=[-1 -1  1  1 -1 -1 -1 -1 -1 -1]}
      mask prompts: edge "Edge Type"; polarity "Output Polarity"; x_in "Input X Positions"; y_in "Input Y Positions"; x_out "Output X Positions"; y_out "Output Y Positions"
      mask help: Output is active for one-cycle after each edge of the specified type (i.e. rising, falling or both).
      mask init: same as mdt_snap_10ch_daq/edge_detect1
      settings: AttributesFormatString=|
      | rising edges
      | active high
      mask Help: Output is active for one-cycle after each edge of the specified type (i.e. rising, falling, or both).  Latency is zero.
      mask TypeOptions edge: Rising | Falling | Both
      mask TypeOptions polarity: Active High | Active Low
      mask Display:
      | plot(x_in_num,0.5+y_in_num*0.2);
      | plot(x_out_num,0.5+y_out_num*0.2);
  edge_detect5 : Subsystem  AncestorBlock=casper_library_misc/edge_detect  mask(edge_detect){edge=Rising, polarity=Active High, x_in=[0 0.08 0.08 0.16 0.16 0.24 0.24 0.32 0.32 0.4], y_in=[-1 -1  1  1  1  1  1  1  1  1], x_out=[0.6 0.68 0.68 0.76 0.76 0.84 0.84 0.92 0.92 1], y_out=[-1 -1  1  1 -1 -1 -1 -1 -1 -1]}
      mask prompts: edge "Edge Type"; polarity "Output Polarity"; x_in "Input X Positions"; y_in "Input Y Positions"; x_out "Output X Positions"; y_out "Output Y Positions"
      mask help: Output is active for one-cycle after each edge of the specified type (i.e. rising, falling or both).
      mask init: same as mdt_snap_10ch_daq/edge_detect1
      settings: AttributesFormatString=|
      | rising edges
      | active high
      mask Help: Output is active for one-cycle after each edge of the specified type (i.e. rising, falling, or both).  Latency is zero.
      mask TypeOptions edge: Rising | Falling | Both
      mask TypeOptions polarity: Active High | Active Low
      mask Display:
      | plot(x_in_num,0.5+y_in_num*0.2);
      | plot(x_out_num,0.5+y_out_num*0.2);
  edge_detect9 : Subsystem  AncestorBlock=casper_library_misc/edge_detect  mask(edge_detect){edge=Rising, polarity=Active High, x_in=[0 0.08 0.08 0.16 0.16 0.24 0.24 0.32 0.32 0.4], y_in=[-1 -1  1  1  1  1  1  1  1  1], x_out=[0.6 0.68 0.68 0.76 0.76 0.84 0.84 0.92 0.92 1], y_out=[-1 -1  1  1 -1 -1 -1 -1 -1 -1]}
      mask prompts: edge "Edge Type"; polarity "Output Polarity"; x_in "Input X Positions"; y_in "Input Y Positions"; x_out "Output X Positions"; y_out "Output Y Positions"
      mask help: Output is active for one-cycle after each edge of the specified type (i.e. rising, falling or both).
      mask init: same as mdt_snap_10ch_daq/edge_detect1
      settings: AttributesFormatString=|
      | rising edges
      | active high
      mask Help: Output is active for one-cycle after each edge of the specified type (i.e. rising, falling, or both).  Latency is zero.
      mask TypeOptions edge: Rising | Falling | Both
      mask TypeOptions polarity: Active High | Active Low
      mask Display:
      | plot(x_in_num,0.5+y_in_num*0.2);
      | plot(x_out_num,0.5+y_out_num*0.2);
  enable_daq : Subsystem  Tag=xps:sw_reg  AncestorBlock=xps_library/Memory/software_register  mask(swreg){io_dir=From Processor, io_delay=0, init_val=0, sample_period=1, names=reg, bitwidths=32, bin_pts=0, arith_types=0, sim_port=on, show_format=on}
      mask prompts: io_dir "I/O direction"; io_delay "I/O delay"; init_val "Initial Value"; sample_period "Sample period"; names "Bitfield names [msb...lsb]"; bitwidths "Bitfield widths"; bin_pts "Bitfield binary pts"; arith_types "Bitfield types, ufix=0, fix=1, bool=2"; sim_port "Provide sim input/output?"; show_format "Print format string?"
      mask help: A 32-bit software-accessible register. Can be divided into bitfields of varying widths and types using the fields in the block mask.
      mask init:
      | swreg_init(gcb)
      settings: AttributesFormatString=1input:uf32.0 = 32 bits
      mask TypeOptions io_dir: To Processor | From Processor
      mask Callback io_dir:
      | mask_enables = get_param(gcb, 'MaskEnables');
      | mask_names = get_param(gcb, 'MaskNames');
      | if strcmp(get_param(gcb, 'io_dir'), 'To Processor'),
      |     mask_enables{ismember(mask_names, 'sample_period')} = 'off';
      | else
      |     mask_enables{ismember(mask_names, 'sample_period')} = 'on';
      | end
      | set_param(gcb, 'MaskEnables', mask_enables);
      mask DialogControl ParameterTabVar0 Prompt: Setup
  gbe0 : Subsystem  Tag=xps:ten_gbe  AncestorBlock=xps_library/IO/ten_gbe  mask(ten_gbe){flavour=sfp+, slot=0, port_r1=0, port_r2_cx4=0, port_r2_sfpp=0, rx_dist_ram=on, large_frames=on, show_param=on, pre_emph_r2=1.07, pre_emph=3, post_emph_r2=0.18, rxeqmix_r2=7, swing_r2=940, swing=800, fab_en=on, fab_mac=hex2dec('123456780000'), fab_ip=172*(2^24) + 22*(2^16) + 37*(2^8) + 31*(2^0), fab_udp=52000, fab_gate=1, cpu_rx_en=on, cpu_tx_en=on, ttl=hex2dec('FF'), promisc_mode=off, debug_ctr_width=32, txctr=on, txerrctr=off, txerrctr_len=100, txofctr=on, txfullctr=on, txvldctr=on, txsnaplen=8192, rxctr=on, rxerrctr=off, rxerrctr_len=100, rxofctr=on, rxbadctr=on, rxvldctr=on, rxeofctr=on, rxsnaplen=8192}
      mask prompts: flavour "Mezzanine card flavour"; slot "Card slot"; port_r1 "Port"; port_r2_cx4 "Port"; port_r2_sfpp "Port"; rx_dist_ram "Shallow RX Fifo (Beware overruns!)"; large_frames "Enable Large TX Frames (8k+512)"; show_param "---------------------- Show Implementation Parameters -----------------------------------------------------------------------------------"; pre_emph_r2 "Pre-emphasis (dB)"; pre_emph "Pre-emphasis"; post_emph_r2 "Post-emphasis (dB)"; rxeqmix_r2 "Receive equalisation"; swing_r2 "Driver Swing Control (mVppd)"; swing "Differential swing"; fab_en "Enable fabric on startup"; fab_mac "Fabric MAC Address"; fab_ip "Fabric IP Address"; fab_udp "Fabric UDP Port"; fab_gate "Fabric Gateway"; cpu_rx_en "Enable CPU RX"; cpu_tx_en "Enable CPU TX"; promisc_mode "Promiscuous mode"; debug_ctr_width "Debug counter width"; txctr "TX - core_txctr"; txerrctr "TX packet length error - core_txerrctr"; txerrctr_len "-- expected TX packet length"; txofctr "TX overflow - core_txofctr"; txfullctr "TX full - core_txfullctr"; txvldctr "TX valid cycle - core_txvldctr"; txsnaplen "TX snapshot length"; rxctr "RX - core_rxctr"; rxerrctr "RX packet length error - core_rxerrctr"; rxerrctr_len "-- expected RX packet length"; rxofctr "RX overflow - core_rxofctr"; rxbadctr "RX bad - core_rxbadctr"; rxvldctr "RX valid cycle - core_rxvldctr"; rxeofctr "RX eof - core_rxeofctr"; rxsnaplen "RX snapshot length"
      mask help: This block sends and receives UDP frames (packets). It accepts a 64 bit wide data stream with user-determined frame breaks. The data stream is wrapped in a UDP frame for transmission. Incoming UDP packets are unwrapped and the data presented as a 64 bit wide stream.
      mask init:
      | temp = eval(get_param(gcb, 'debug_ctr_width'));
      | if temp <= 0,
      |     error('Debug counters cannot be ltoet zero.');
      | end
      | tengbe_mask(gcb)
      mask TypeOptions flavour: sfp+ | cx4
      mask Callback flavour: tengbe_callback
      mask TypeOptions slot: 0 | 1
      mask TypeOptions port_r1: 0 | 1 | 2 | 3
      mask TypeOptions port_r2_cx4: 0 | 1 | 2
      mask TypeOptions port_r2_sfpp: 0 | 1 | 2 | 3
      mask Callback show_param: tengbe_callback
      mask TypeOptions pre_emph_r2: 0.15 | 0.3 | 0.45 | 0.61 | 0.74 | 0.91 | 1.07 | 1.25 | 1.36 | 1.55 | 1.74 | 1.94 | 2.11 | 2.32 | 2.54 | 2.77
      mask TypeOptions pre_emph: 0 | 1 | 2 | 3
      mask TypeOptions post_emph_r2: 0.18 | 0.19 | 0.2 | 0.39 | 0.63 | 0.82 | 1.07 | 1.32 | 1.6 | 1.65 | 1.94 | 2.21 | 2.52 | 2.76 | 3.08 | 3.41 | 3.77 | 3.97 | 4.36 | 4.73 | 5.16 | 5.47 | 5.93 | 6.38 | 6.89
      mask TypeOptions rxeqmix_r2: 0 | 1 | 2 | 3 | 4 | 5 | 6 | 7
      mask TypeOptions swing_r2: 110 | 210 | 310 | 400 | 480 | 570 | 660 | 740 | 810 | 880 | 940 | 990 | 1040 | 1080 | 1110 | 1130
      mask TypeOptions swing: 400 | 500 | 600 | 700 | 800
      mask Callback txerrctr:
      | blk = gcb;
      | mask_visibilities = get_param(blk, 'MaskVisibilities');
      | mask_names = get_param(blk, 'MaskNames');
      | if strcmp(get_param(blk, 'txerrctr'), 'on')
      |     mask_visibilities{ismember(mask_names, 'txerrctr_len')} = 'on';
      | else
      |     mask_visibilities{ismember(mask_names, 'txerrctr_len')} = 'off';
      | end
      | set_param(blk, 'MaskVisibilities', mask_visibilities);
      mask TypeOptions txsnaplen: 0 - no snap | 256 | 512 | 1024 | 2048 | 4096 | 8192 | 16384
      mask Callback rxerrctr:
      | blk = gcb;
      | mask_visibilities = get_param(blk, 'MaskVisibilities');
      | mask_names = get_param(blk, 'MaskNames');
      | if strcmp(get_param(blk, 'rxerrctr'), 'on')
      |     mask_visibilities{ismember(mask_names, 'rxerrctr_len')} = 'on';
      | else
      |     mask_visibilities{ismember(mask_names, 'rxerrctr_len')} = 'off';
      | end
      | set_param(blk, 'MaskVisibilities', mask_visibilities);
      mask TypeOptions rxsnaplen: 0 - no snap | 256 | 512 | 1024 | 2048 | 4096 | 8192 | 16384
      mask DialogControl ParameterTabVar0 Prompt: Core
      mask DialogControl ParameterTabVar01 Prompt: Debug counters
  led0 : xps_library/IO/gpio  Tag=xps:gpio  io_group_params_forwarded=off  io_group=ROACH:led  io_group_real=led  io_group_custom=0  io_dir=out  arith_type=Boolean  bitwidth=1  bin_pt=0  bit_index=0  sample_period=1  use_single_ended=off  use_ddr=off  reg_iob=on  reg_clk_phase=0  termination=None
      settings: SourceProductName=CASPER XPS Blockset
  led1 : xps_library/IO/gpio  Tag=xps:gpio  io_group_params_forwarded=off  io_group=ROACH:led  io_group_real=led  io_group_custom=0  io_dir=out  arith_type=Boolean  bitwidth=1  bin_pt=0  bit_index=1  sample_period=1  use_single_ended=off  use_ddr=off  reg_iob=on  reg_clk_phase=0  termination=None
      settings: SourceProductName=CASPER XPS Blockset
  led2 : xps_library/IO/gpio  Tag=xps:gpio  io_group_params_forwarded=off  io_group=ROACH:led  io_group_real=led  io_group_custom=0  io_dir=out  arith_type=Boolean  bitwidth=1  bin_pt=0  bit_index=2  sample_period=1  use_single_ended=off  use_ddr=off  reg_iob=on  reg_clk_phase=0  termination=None
      settings: SourceProductName=CASPER XPS Blockset
  led3 : xps_library/IO/gpio  Tag=xps:gpio  io_group_params_forwarded=off  io_group=ROACH:led  io_group_real=led  io_group_custom=0  io_dir=out  arith_type=Boolean  bitwidth=1  bin_pt=0  bit_index=3  sample_period=1  use_single_ended=off  use_ddr=off  reg_iob=on  reg_clk_phase=0  termination=None
      settings: SourceProductName=CASPER XPS Blockset
  mixer1 : Subsystem  Tag=casper:mixer  AncestorBlock=casper_library_downconverter/mixer  mask(mixer){freq_div=32768, freq=10145, nstreams=1, n_bits=8, bram_latency=2, mult_latency=4}
      mask prompts: freq_div "Frequency Divisions (M)"; freq "Mixing Frequency (? / M*2pi)"; nstreams "Number of Parallel Streams"; n_bits "Bit Width"; bram_latency "BRAM Latency"; mult_latency "Mult Latency"
      mask help: Digitally mixes an input signal (which can be several samples in parallel) with an LO of the indicated frequency (which is some fraction of the native FPGA clock rate).
      mask init:
      | mixer_init(gcb, ...
      |     'freq_div', freq_div, ...
      |     'freq', freq, ...
      |     'nstreams', nstreams, ...
      |     'n_bits', n_bits, ...
      |     'bram_latency', bram_latency, ...
      |     'mult_latency', mult_latency);
      settings: AttributesFormatString=lo at -10145/32768
  mixer10 : Subsystem  Tag=casper:mixer  AncestorBlock=casper_library_downconverter/mixer  mask(mixer){freq_div=32768, freq=10145, nstreams=1, n_bits=8, bram_latency=2, mult_latency=4}
      mask prompts: freq_div "Frequency Divisions (M)"; freq "Mixing Frequency (? / M*2pi)"; nstreams "Number of Parallel Streams"; n_bits "Bit Width"; bram_latency "BRAM Latency"; mult_latency "Mult Latency"
      mask help: Digitally mixes an input signal (which can be several samples in parallel) with an LO of the indicated frequency (which is some fraction of the native FPGA clock rate).
      mask init: same as mdt_snap_10ch_daq/mixer1
      settings: AttributesFormatString=lo at -10145/32768
  mixer2 : Subsystem  Tag=casper:mixer  AncestorBlock=casper_library_downconverter/mixer  mask(mixer){freq_div=32768, freq=10145, nstreams=1, n_bits=8, bram_latency=2, mult_latency=4}
      mask prompts: freq_div "Frequency Divisions (M)"; freq "Mixing Frequency (? / M*2pi)"; nstreams "Number of Parallel Streams"; n_bits "Bit Width"; bram_latency "BRAM Latency"; mult_latency "Mult Latency"
      mask help: Digitally mixes an input signal (which can be several samples in parallel) with an LO of the indicated frequency (which is some fraction of the native FPGA clock rate).
      mask init: same as mdt_snap_10ch_daq/mixer1
      settings: AttributesFormatString=lo at -10145/32768
  mixer3 : Subsystem  Tag=casper:mixer  AncestorBlock=casper_library_downconverter/mixer  mask(mixer){freq_div=32768, freq=10145, nstreams=1, n_bits=8, bram_latency=2, mult_latency=4}
      mask prompts: freq_div "Frequency Divisions (M)"; freq "Mixing Frequency (? / M*2pi)"; nstreams "Number of Parallel Streams"; n_bits "Bit Width"; bram_latency "BRAM Latency"; mult_latency "Mult Latency"
      mask help: Digitally mixes an input signal (which can be several samples in parallel) with an LO of the indicated frequency (which is some fraction of the native FPGA clock rate).
      mask init: same as mdt_snap_10ch_daq/mixer1
      settings: AttributesFormatString=lo at -10145/32768
  mixer4 : Subsystem  Tag=casper:mixer  AncestorBlock=casper_library_downconverter/mixer  mask(mixer){freq_div=32768, freq=10145, nstreams=1, n_bits=8, bram_latency=2, mult_latency=4}
      mask prompts: freq_div "Frequency Divisions (M)"; freq "Mixing Frequency (? / M*2pi)"; nstreams "Number of Parallel Streams"; n_bits "Bit Width"; bram_latency "BRAM Latency"; mult_latency "Mult Latency"
      mask help: Digitally mixes an input signal (which can be several samples in parallel) with an LO of the indicated frequency (which is some fraction of the native FPGA clock rate).
      mask init: same as mdt_snap_10ch_daq/mixer1
      settings: AttributesFormatString=lo at -10145/32768
  mixer5 : Subsystem  Tag=casper:mixer  AncestorBlock=casper_library_downconverter/mixer  mask(mixer){freq_div=32768, freq=10145, nstreams=1, n_bits=8, bram_latency=2, mult_latency=4}
      mask prompts: freq_div "Frequency Divisions (M)"; freq "Mixing Frequency (? / M*2pi)"; nstreams "Number of Parallel Streams"; n_bits "Bit Width"; bram_latency "BRAM Latency"; mult_latency "Mult Latency"
      mask help: Digitally mixes an input signal (which can be several samples in parallel) with an LO of the indicated frequency (which is some fraction of the native FPGA clock rate).
      mask init: same as mdt_snap_10ch_daq/mixer1
      settings: AttributesFormatString=lo at -10145/32768
  mixer6 : Subsystem  Tag=casper:mixer  AncestorBlock=casper_library_downconverter/mixer  mask(mixer){freq_div=32768, freq=10145, nstreams=1, n_bits=8, bram_latency=2, mult_latency=4}
      mask prompts: freq_div "Frequency Divisions (M)"; freq "Mixing Frequency (? / M*2pi)"; nstreams "Number of Parallel Streams"; n_bits "Bit Width"; bram_latency "BRAM Latency"; mult_latency "Mult Latency"
      mask help: Digitally mixes an input signal (which can be several samples in parallel) with an LO of the indicated frequency (which is some fraction of the native FPGA clock rate).
      mask init: same as mdt_snap_10ch_daq/mixer1
      settings: AttributesFormatString=lo at -10145/32768
  mixer7 : Subsystem  Tag=casper:mixer  AncestorBlock=casper_library_downconverter/mixer  mask(mixer){freq_div=32768, freq=10145, nstreams=1, n_bits=8, bram_latency=2, mult_latency=4}
      mask prompts: freq_div "Frequency Divisions (M)"; freq "Mixing Frequency (? / M*2pi)"; nstreams "Number of Parallel Streams"; n_bits "Bit Width"; bram_latency "BRAM Latency"; mult_latency "Mult Latency"
      mask help: Digitally mixes an input signal (which can be several samples in parallel) with an LO of the indicated frequency (which is some fraction of the native FPGA clock rate).
      mask init: same as mdt_snap_10ch_daq/mixer1
      settings: AttributesFormatString=lo at -10145/32768
  mixer8 : Subsystem  Tag=casper:mixer  AncestorBlock=casper_library_downconverter/mixer  mask(mixer){freq_div=32768, freq=10145, nstreams=1, n_bits=8, bram_latency=2, mult_latency=4}
      mask prompts: freq_div "Frequency Divisions (M)"; freq "Mixing Frequency (? / M*2pi)"; nstreams "Number of Parallel Streams"; n_bits "Bit Width"; bram_latency "BRAM Latency"; mult_latency "Mult Latency"
      mask help: Digitally mixes an input signal (which can be several samples in parallel) with an LO of the indicated frequency (which is some fraction of the native FPGA clock rate).
      mask init: same as mdt_snap_10ch_daq/mixer1
      settings: AttributesFormatString=lo at -10145/32768
  mixer9 : Subsystem  Tag=casper:mixer  AncestorBlock=casper_library_downconverter/mixer  mask(mixer){freq_div=32768, freq=10145, nstreams=1, n_bits=8, bram_latency=2, mult_latency=4}
      mask prompts: freq_div "Frequency Divisions (M)"; freq "Mixing Frequency (? / M*2pi)"; nstreams "Number of Parallel Streams"; n_bits "Bit Width"; bram_latency "BRAM Latency"; mult_latency "Mult Latency"
      mask help: Digitally mixes an input signal (which can be several samples in parallel) with an LO of the indicated frequency (which is some fraction of the native FPGA clock rate).
      mask init: same as mdt_snap_10ch_daq/mixer1
      settings: AttributesFormatString=lo at -10145/32768
  pipeline1 : Subsystem  AncestorBlock=casper_library_delays/pipeline  mask(pipeline){csp_latency=2}
      mask prompts: csp_latency "Latency"
      mask help:
      | An explicitly laid-out delay line to avoid mapping to SRL16s
      | for use in pipelining to help achieve timing closure.
      mask init:
      | pipeline_init(gcb,'latency',csp_latency);
      settings: AttributesFormatString=Latency = %<latency>
      mask Display:
      | port_label('input', 1, 'd');
      | port_label('output', 1, 'q');
      | disp(['Z^-', num2str(csp_latency)]);
  pipeline12 : Subsystem  AncestorBlock=casper_library_delays/pipeline  mask(pipeline){csp_latency=1}
      mask prompts: csp_latency "Latency"
      mask help:
      | An explicitly laid-out delay line to avoid mapping to SRL16s
      | for use in pipelining to help achieve timing closure.
      mask init:
      | pipeline_init(gcb,'latency',csp_latency);
      settings: AttributesFormatString=Latency = %<latency>
      mask Display:
      | port_label('input', 1, 'd');
      | port_label('output', 1, 'q');
      | disp(['Z^-', num2str(csp_latency)]);
  pipeline2 : Subsystem  AncestorBlock=casper_library_delays/pipeline  mask(pipeline){csp_latency=4}
      mask prompts: csp_latency "Latency"
      mask help:
      | An explicitly laid-out delay line to avoid mapping to SRL16s
      | for use in pipelining to help achieve timing closure.
      mask init:
      | pipeline_init(gcb,'latency',csp_latency);
      settings: AttributesFormatString=Latency = %<latency>
      mask Display:
      | port_label('input', 1, 'd');
      | port_label('output', 1, 'q');
      | disp(['Z^-', num2str(csp_latency)]);
  pipeline3 : Subsystem  AncestorBlock=casper_library_delays/pipeline  mask(pipeline){csp_latency=3}
      mask prompts: csp_latency "Latency"
      mask help:
      | An explicitly laid-out delay line to avoid mapping to SRL16s
      | for use in pipelining to help achieve timing closure.
      mask init:
      | pipeline_init(gcb,'latency',csp_latency);
      settings: AttributesFormatString=Latency = %<latency>
      mask Display:
      | port_label('input', 1, 'd');
      | port_label('output', 1, 'q');
      | disp(['Z^-', num2str(csp_latency)]);
  pipeline4 : Subsystem  AncestorBlock=casper_library_delays/pipeline  mask(pipeline){csp_latency=6}
      mask prompts: csp_latency "Latency"
      mask help:
      | An explicitly laid-out delay line to avoid mapping to SRL16s
      | for use in pipelining to help achieve timing closure.
      mask init:
      | pipeline_init(gcb,'latency',csp_latency);
      settings: AttributesFormatString=Latency = %<latency>
      mask Display:
      | port_label('input', 1, 'd');
      | port_label('output', 1, 'q');
      | disp(['Z^-', num2str(csp_latency)]);
  pipeline5 : Subsystem  AncestorBlock=casper_library_delays/pipeline  mask(pipeline){csp_latency=5}
      mask prompts: csp_latency "Latency"
      mask help:
      | An explicitly laid-out delay line to avoid mapping to SRL16s
      | for use in pipelining to help achieve timing closure.
      mask init:
      | pipeline_init(gcb,'latency',csp_latency);
      settings: AttributesFormatString=Latency = %<latency>
      mask Display:
      | port_label('input', 1, 'd');
      | port_label('output', 1, 'q');
      | disp(['Z^-', num2str(csp_latency)]);
  pipeline6 : Subsystem  AncestorBlock=casper_library_delays/pipeline  mask(pipeline){csp_latency=8}
      mask prompts: csp_latency "Latency"
      mask help:
      | An explicitly laid-out delay line to avoid mapping to SRL16s
      | for use in pipelining to help achieve timing closure.
      mask init:
      | pipeline_init(gcb,'latency',csp_latency);
      settings: AttributesFormatString=Latency = %<latency>
      mask Display:
      | port_label('input', 1, 'd');
      | port_label('output', 1, 'q');
      | disp(['Z^-', num2str(csp_latency)]);
  pipeline7 : Subsystem  AncestorBlock=casper_library_delays/pipeline  mask(pipeline){csp_latency=7}
      mask prompts: csp_latency "Latency"
      mask help:
      | An explicitly laid-out delay line to avoid mapping to SRL16s
      | for use in pipelining to help achieve timing closure.
      mask init:
      | pipeline_init(gcb,'latency',csp_latency);
      settings: AttributesFormatString=Latency = %<latency>
      mask Display:
      | port_label('input', 1, 'd');
      | port_label('output', 1, 'q');
      | disp(['Z^-', num2str(csp_latency)]);
  pipeline8 : Subsystem  AncestorBlock=casper_library_delays/pipeline  mask(pipeline){csp_latency=10}
      mask prompts: csp_latency "Latency"
      mask help:
      | An explicitly laid-out delay line to avoid mapping to SRL16s
      | for use in pipelining to help achieve timing closure.
      mask init:
      | pipeline_init(gcb,'latency',csp_latency);
      settings: AttributesFormatString=Latency = %<latency>
      mask Display:
      | port_label('input', 1, 'd');
      | port_label('output', 1, 'q');
      | disp(['Z^-', num2str(csp_latency)]);
  pipeline9 : Subsystem  AncestorBlock=casper_library_delays/pipeline  mask(pipeline){csp_latency=9}
      mask prompts: csp_latency "Latency"
      mask help:
      | An explicitly laid-out delay line to avoid mapping to SRL16s
      | for use in pipelining to help achieve timing closure.
      mask init:
      | pipeline_init(gcb,'latency',csp_latency);
      settings: AttributesFormatString=Latency = %<latency>
      mask Display:
      | port_label('input', 1, 'd');
      | port_label('output', 1, 'q');
      | disp(['Z^-', num2str(csp_latency)]);
  pps : xps_library/IO/gpio  Tag=xps:gpio  io_group_params_forwarded=off  io_group=ROACH:led  io_group_real=sync_in  io_group_custom=0  io_dir=in  arith_type=Boolean  bitwidth=1  bin_pt=0  bit_index=0  sample_period=1  use_single_ended=off  use_ddr=off  reg_iob=on  reg_clk_phase=0  termination=None
      settings: SourceProductName=CASPER XPS Blockset
  pulse_ext2 : Subsystem  AncestorBlock=casper_library_misc/pulse_ext  mask(pulse_ext){pulse_len=2^24}
      mask prompts: pulse_len "Length of Pulse"
      mask help:
      | Extends a boolean signal to be high for the specified number of clocks after
      | the last high input.
      mask init:
      | bits = ceil(log2(pulse_len+1));
      mask Help: eval('xlWeb(''http://casper.berkeley.edu/wiki/Pulse_ext'')')
  reset_gbe0 : Subsystem  Tag=xps:sw_reg  AncestorBlock=xps_library/Memory/software_register  mask(swreg){io_dir=From Processor, io_delay=0, init_val=0, sample_period=1, names=reg, bitwidths=32, bin_pts=0, arith_types=0, sim_port=on, show_format=on}
      mask prompts: io_dir "I/O direction"; io_delay "I/O delay"; init_val "Initial Value"; sample_period "Sample period"; names "Bitfield names [msb...lsb]"; bitwidths "Bitfield widths"; bin_pts "Bitfield binary pts"; arith_types "Bitfield types, ufix=0, fix=1, bool=2"; sim_port "Provide sim input/output?"; show_format "Print format string?"
      mask help: A 32-bit software-accessible register. Can be divided into bitfields of varying widths and types using the fields in the block mask.
      mask init:
      | swreg_init(gcb)
      settings: AttributesFormatString=1input:uf32.0 = 32 bits
      mask TypeOptions io_dir: To Processor | From Processor
      mask Callback io_dir:
      | mask_enables = get_param(gcb, 'MaskEnables');
      | mask_names = get_param(gcb, 'MaskNames');
      | if strcmp(get_param(gcb, 'io_dir'), 'To Processor'),
      |     mask_enables{ismember(mask_names, 'sample_period')} = 'off';
      | else
      |     mask_enables{ismember(mask_names, 'sample_period')} = 'on';
      | end
      | set_param(gcb, 'MaskEnables', mask_enables);
      mask DialogControl ParameterTabVar0 Prompt: Setup
  reset_pktIdx : Subsystem  Tag=xps:sw_reg  AncestorBlock=xps_library/Memory/software_register  mask(swreg){io_dir=From Processor, io_delay=0, init_val=0, sample_period=1, names=reg, bitwidths=32, bin_pts=0, arith_types=0, sim_port=on, show_format=on}
      mask prompts: io_dir "I/O direction"; io_delay "I/O delay"; init_val "Initial Value"; sample_period "Sample period"; names "Bitfield names [msb...lsb]"; bitwidths "Bitfield widths"; bin_pts "Bitfield binary pts"; arith_types "Bitfield types, ufix=0, fix=1, bool=2"; sim_port "Provide sim input/output?"; show_format "Print format string?"
      mask help: A 32-bit software-accessible register. Can be divided into bitfields of varying widths and types using the fields in the block mask.
      mask init:
      | swreg_init(gcb)
      settings: AttributesFormatString=1input:uf32.0 = 32 bits
      mask TypeOptions io_dir: To Processor | From Processor
      mask Callback io_dir:
      | mask_enables = get_param(gcb, 'MaskEnables');
      | mask_names = get_param(gcb, 'MaskNames');
      | if strcmp(get_param(gcb, 'io_dir'), 'To Processor'),
      |     mask_enables{ismember(mask_names, 'sample_period')} = 'off';
      | else
      |     mask_enables{ismember(mask_names, 'sample_period')} = 'on';
      | end
      | set_param(gcb, 'MaskEnables', mask_enables);
      mask DialogControl ParameterTabVar0 Prompt: Setup
  snapIdx : Subsystem  Tag=xps:sw_reg  AncestorBlock=xps_library/Memory/software_register  mask(swreg){io_dir=From Processor, io_delay=0, init_val=0, sample_period=1, names=reg, bitwidths=32, bin_pts=0, arith_types=0, sim_port=on, show_format=on}
      mask prompts: io_dir "I/O direction"; io_delay "I/O delay"; init_val "Initial Value"; sample_period "Sample period"; names "Bitfield names [msb...lsb]"; bitwidths "Bitfield widths"; bin_pts "Bitfield binary pts"; arith_types "Bitfield types, ufix=0, fix=1, bool=2"; sim_port "Provide sim input/output?"; show_format "Print format string?"
      mask help: A 32-bit software-accessible register. Can be divided into bitfields of varying widths and types using the fields in the block mask.
      mask init:
      | swreg_init(gcb)
      settings: AttributesFormatString=1input:uf32.0 = 32 bits
      mask TypeOptions io_dir: To Processor | From Processor
      mask Callback io_dir:
      | mask_enables = get_param(gcb, 'MaskEnables');
      | mask_names = get_param(gcb, 'MaskNames');
      | if strcmp(get_param(gcb, 'io_dir'), 'To Processor'),
      |     mask_enables{ismember(mask_names, 'sample_period')} = 'off';
      | else
      |     mask_enables{ismember(mask_names, 'sample_period')} = 'on';
      | end
      | set_param(gcb, 'MaskEnables', mask_enables);
      mask DialogControl ParameterTabVar0 Prompt: Setup
  snap_adc : Subsystem  Tag=xps:snap_adc  AncestorBlock=xps_library/ADCs/snap_adc  mask(adc_snap){sample_rate=250, snap_inputs=12, adc_resolution=8}
      mask prompts: sample_rate "Sample rate (MHz)"; snap_inputs "Number of inputs per snap"; adc_resolution "Resolution of ADC (number of bit)"
      mask help: Interface to the 3 adc chips on the SNAP board. Please see Help for instructions on parameter settings
      mask init:
      | adc_snap_init(gcb);
      mask Help:
      | This is the CASPER "yellow block" for the ADCs on the SNAP board.
      | Each ADC chip accepts four inputs.
      | 
      | Maximum sample rate f (Mega samples per second)
      | 
      | Number of inputs         3                6                12
      | Resolution 8 bits          f=1000      f=500         f=250
      | Resolution 12 bits        f=640        f=320         f=160
      | 
      | Resolution 12 bits is available when SNAP board is upgraded with HMCAD1520 ADC chips
      mask TypeOptions snap_inputs: 3 | 6 | 12
      mask TypeOptions adc_resolution: 8 | 12
  stationIdx : Subsystem  Tag=xps:sw_reg  AncestorBlock=xps_library/Memory/software_register  mask(swreg){io_dir=From Processor, io_delay=0, init_val=0, sample_period=1, names=reg, bitwidths=32, bin_pts=0, arith_types=0, sim_port=on, show_format=on}
      mask prompts: io_dir "I/O direction"; io_delay "I/O delay"; init_val "Initial Value"; sample_period "Sample period"; names "Bitfield names [msb...lsb]"; bitwidths "Bitfield widths"; bin_pts "Bitfield binary pts"; arith_types "Bitfield types, ufix=0, fix=1, bool=2"; sim_port "Provide sim input/output?"; show_format "Print format string?"
      mask help: A 32-bit software-accessible register. Can be divided into bitfields of varying widths and types using the fields in the block mask.
      mask init:
      | swreg_init(gcb)
      settings: AttributesFormatString=1input:uf32.0 = 32 bits
      mask TypeOptions io_dir: To Processor | From Processor
      mask Callback io_dir:
      | mask_enables = get_param(gcb, 'MaskEnables');
      | mask_names = get_param(gcb, 'MaskNames');
      | if strcmp(get_param(gcb, 'io_dir'), 'To Processor'),
      |     mask_enables{ismember(mask_names, 'sample_period')} = 'off';
      | else
      |     mask_enables{ismember(mask_names, 'sample_period')} = 'on';
      | end
      | set_param(gcb, 'MaskEnables', mask_enables);
      mask DialogControl ParameterTabVar0 Prompt: Setup
  sync_gen : Subsystem  AncestorBlock=casper_library_misc/sync_gen  mask(sync_gen){sim_acc_len=1, fft_size=1, fft_simult_inputs=1, pfb_fir_taps=1, reorder_vec=1, scale=1}
      mask prompts: sim_acc_len "Simulation Accumulation Length"; fft_size "FFT Size"; fft_simult_inputs "Simultaneous Inputs (FFT)"; pfb_fir_taps "Taps in pfb_fir (use 1 if no pfb_fir)"; reorder_vec "Reorder Orders (e.g. [2 2 2])"
      mask help:
      | This block computes the sync period based on system parameters as
      | described in Casper memo.  Detailed descritions of the block's
      | variables can be found in the 'Block Documentation' section of
      | the CASPER wiki.
      mask init:
      | sync_gen_init(gcb, ...
      |     'sim_acc_len', sim_acc_len, ...
      |     'fft_size', fft_size, ...
      |     'fft_simult_inputs', fft_simult_inputs,...
      |     'pfb_fir_taps', pfb_fir_taps, ...
      |     'reorder_vec', reorder_vec, ...
      |     'scale', scale);
      settings: AttributesFormatString=sim_sync_period=1
      mask Help:
      | SyncPeriod=LCM(reorder_vec)*(acc_num)*(pfb_fir_len)*(fft_size/fft_simult_inputs)
      | 
      | See CASPER sync pulse memo for more details.
  wires:
  [eth_valid] -> Register28/1
  Counter3/1 -> Relational2/1
  Constant/1 -> Relational2/2
  Mux4/1 -> Register29/1
  Constant105/1 -> stationIdx/1(sim_1)
  Constant106/1 -> snapIdx/1(sim_1)
  Constant108/1 -> Nelements/1(sim_1)
  Constant109/1 -> SperElement/1(sim_1)
  stationIdx/1(in_reg) -> [stationIdx]
  snapIdx/1(in_reg) -> [snapIdx]
  Nelements/1(in_reg) -> [Nelements]
  SperElement/1(in_reg) -> [SperElement]
  BitBasher1/1 -> Mux4/2
  [new_pkt] -> Counter10/1
  [ch_valid] -> edge_detect4/1(in)
  edge_detect4/1(out) -> Counter10/2
  [SperElement] -> Relational10/1
  Counter10/1 -> Relational10/2
  [ch_last] -> Logical2/1
  Relational10/1 -> Logical2/2
  Logical2/1 -> [end_pkt], edge_detect5/1(in)
  Logical4/1 -> [new_pkt]
  Counter7/1 -> Relational12/2, Relational13/2, [channelIdx]
  Constant110/1 -> AddSub1/2
  AddSub1/1 -> Relational13/1
  [new_pkt] -> Counter6/1
  Counter6/1 -> [contentIdx], Relational11/2
  Constant3/1 -> Relational11/1
  Relational11/1 -> [hdr_valid], Counter6/2
  Logical5/1 -> Counter7/2
  [hdr_valid] -> Inverter1/1
  [contentIdx] -> Mux4/1
  [end_pkt] -> Counter2/2
  [reset_pktIdx] -> Counter2/1
  Counter2/1 -> [packetIdx]
  Relational2/1 -> Counter3/1, [dec_clk]
  [Nelements] -> Relational12/1, AddSub1/1
  Relational13/1 -> [ch_last]
  edge_detect5/1(out) -> Delay2/1
  [reset_pktcnt] -> Logical4/2
  Delay2/1 -> Logical4/1
  Relational12/1 -> Logical5/3, Logical6/1
  [enable_pkt] -> Logical5/2
  Inverter1/1 -> Logical5/1
  Logical10/1 -> Logical3/2
  [enable_pkt] -> Logical3/1
  [hdr_valid] -> Logical10/1
  [ch_valid] -> Logical10/2
  [dec_clk] -> Counter7/1
  [enable_pkt] -> Logical6/2
  Constant111/1 -> Mux5/2
  Logical6/1 -> Mux5/3
  Logical7/1 -> Counter11/2
  [dec_clk] -> Logical7/1
  Inverter3/1 -> Logical7/2
  [new_pkt] -> Counter11/1
  Mux5/1 -> [ch_valid]
  Counter11/1 -> Mux5/1, Convert1/1
  Convert1/1 -> Inverter3/1
  led0/1 -> Terminator3/1
  [enable_pkt] -> Register1/1
  [eth_valid] -> Register55/1
  Register1/1 -> led0/1
  led2/1 -> Terminator7/1
  Register55/1 -> led2/1
  edge_detect9/1(out) -> [reset_pktcnt]
  Register2/1 -> Slice4/1
  enable_daq/1(in_reg) -> Register2/1
  Constant114/1 -> enable_daq/1(sim_1)
  Delay4/1 -> [enable_pkt]
  [snapIdx] -> BitBasher1/2
  [stationIdx] -> BitBasher1/1
  [packetIdx] -> BitBasher2/1
  Constant107/1 -> BitBasher2/2
  BitBasher2/1 -> Mux4/3
  Constant2/1 -> reset_pktIdx/1(sim_1)
  Register3/1 -> Slice1/1
  reset_pktIdx/1(in_reg) -> Register3/1
  Slice1/1 -> [reset_pktIdx]
  Band-Limited White Noise/1 -> snap_adc/1(a1_sim), snap_adc/2(a2_sim), snap_adc/3(a3_sim), snap_adc/4(a4_sim), snap_adc/5(b1_sim), snap_adc/6(b2_sim), snap_adc/12(c4_sim), snap_adc/11(c3_sim), snap_adc/10(c2_sim), snap_adc/9(c1_sim), snap_adc/8(b4_sim), snap_adc/7(b3_sim)
  Reinterpret32/1 -> Convert3/1
  mixer3/1(sync_out) -> Terminator9/1
  Shift2/1 -> Reinterpret32/1
  mixer2/3(imag1) -> Register5/1
  Reinterpret36/1 -> Convert5/1
  Shift4/1 -> Reinterpret36/1
  mixer1/1(sync_out) -> Terminator28/1
  Register4/1 -> mixer1/2(din1)
  Reinterpret34/1 -> Convert/1
  mixer1/3(imag1) -> Register11/1
  Shift9/1 -> Reinterpret37/1
  sync_gen/1(sync_out) -> Register10/1
  mixer3/3(imag1) -> Register9/1
  mixer3/2(real1) -> Register13/1
  mixer1/2(real1) -> Register6/1
  mixer2/2(real1) -> Register8/1
  Register7/1 -> mixer2/2(din1)
  Reinterpret37/1 -> Convert10/1
  mixer2/1(sync_out) -> Terminator8/1
  Register12/1 -> mixer3/2(din1)
  Shift/1 -> Reinterpret34/1
  Register14/1 -> mixer4/2(din1)
  mixer4/2(real1) -> Register15/1
  mixer4/3(imag1) -> Register16/1
  mixer4/1(sync_out) -> Terminator1/1
  mixer8/1(sync_out) -> Terminator2/1
  mixer8/3(imag1) -> Register22/1
  mixer8/2(real1) -> Register21/1
  Register20/1 -> mixer8/2(din1)
  Register18/1 -> mixer7/2(din1)
  mixer6/1(sync_out) -> Terminator5/1
  Register26/1 -> mixer6/2(din1)
  mixer6/2(real1) -> Register27/1
  mixer5/2(real1) -> Register25/1
  mixer7/2(real1) -> Register19/1
  mixer7/3(imag1) -> Register31/1
  mixer5/3(imag1) -> Register17/1
  Register23/1 -> mixer5/2(din1)
  mixer5/1(sync_out) -> Terminator4/1
  mixer6/3(imag1) -> Register24/1
  mixer7/1(sync_out) -> Terminator11/1
  mixer10/3(imag1) -> Register39/1
  mixer9/1(sync_out) -> Terminator17/1
  Register38/1 -> mixer9/2(din1)
  mixer9/3(imag1) -> Register32/1
  Register10/1 -> mixer10/1(sync), mixer9/1(sync), mixer8/1(sync), mixer7/1(sync), mixer6/1(sync), mixer5/1(sync), mixer4/1(sync), mixer3/1(sync), mixer2/1(sync), mixer1/1(sync)
  mixer9/2(real1) -> Register40/1
  mixer10/2(real1) -> Register42/1
  Register41/1 -> mixer10/2(din1)
  mixer10/1(sync_out) -> Terminator19/1
  snap_adc/1(a1) -> Register4/1
  snap_adc/2(a2) -> Register7/1
  snap_adc/3(a3) -> Register12/1
  snap_adc/4(a4) -> Register14/1
  snap_adc/5(b1) -> Register23/1
  snap_adc/6(b2) -> Register26/1
  snap_adc/7(b3) -> Register18/1
  snap_adc/8(b4) -> Register20/1
  snap_adc/10(c2) -> Register41/1
  snap_adc/9(c1) -> Register38/1
  Stage1_ch1-6/3 -> Shift/1
  Stage1_ch1-6/4 -> Shift1/1
  Shift1/1 -> Reinterpret12/1
  Reinterpret12/1 -> Convert2/1
  Reinterpret13/1 -> Convert4/1
  Shift3/1 -> Reinterpret13/1
  Stage1_ch1-6/5 -> Shift3/1
  Stage1_ch1-6/8 -> Shift7/1
  Shift7/1 -> Reinterpret15/1
  Reinterpret15/1 -> Convert9/1
  Reinterpret14/1 -> Convert8/1
  Shift6/1 -> Reinterpret14/1
  Stage1_ch1-6/7 -> Shift6/1
  Stage1_ch1-6/6 -> Shift5/1
  Shift5/1 -> Reinterpret16/1
  Reinterpret16/1 -> Convert6/1
  Reinterpret21/1 -> Convert28/1
  Shift27/1 -> Reinterpret21/1
  Stage1_ch1-6/12 -> Shift27/1
  Stage1_ch1-6/13 -> Shift28/1
  Shift28/1 -> Reinterpret19/1
  Reinterpret19/1 -> Convert29/1
  Reinterpret20/1 -> Convert30/1
  Shift29/1 -> Reinterpret20/1
  Stage1_ch1-6/14 -> Shift29/1
  Stage1_ch1-6/11 -> Shift26/1
  Shift26/1 -> Reinterpret18/1
  Reinterpret18/1 -> Convert27/1
  Reinterpret17/1 -> Convert26/1
  Shift10/1 -> Reinterpret17/1
  Stage1_ch1-6/10 -> Shift10/1
  Stage1_ch1-6/9 -> Shift8/1
  Shift8/1 -> Reinterpret22/1
  Reinterpret22/1 -> Convert25/1
  Register6/1 -> Stage1_ch1-6/1
  Register11/1 -> Stage1_ch1-6/2
  Reinterpret51/1 -> Convert33/1
  Shift41/1 -> Reinterpret51/1
  Stage1_ch7-10/9 -> Shift41/1
  Stage1_ch7-10/10 -> Shift32/1
  Shift32/1 -> Reinterpret33/1
  Reinterpret33/1 -> Convert34/1
  Reinterpret31/1 -> Convert40/1
  Shift38/1 -> Reinterpret31/1
  Stage1_ch7-10/6 -> Shift38/1
  Stage1_ch7-10/7 -> Shift39/1
  Shift39/1 -> Reinterpret29/1
  Reinterpret29/1 -> Convert41/1
  Reinterpret30/1 -> Convert42/1
  Shift40/1 -> Reinterpret30/1
  Stage1_ch7-10/8 -> Shift40/1
  Stage1_ch7-10/5 -> Shift37/1
  Shift37/1 -> Reinterpret24/1
  Reinterpret24/1 -> Convert39/1
  Reinterpret23/1 -> Convert32/1
  Shift31/1 -> Reinterpret23/1
  Stage1_ch7-10/4 -> Shift31/1
  Stage1_ch7-10/3 -> Shift30/1
  Shift30/1 -> Reinterpret52/1
  Reinterpret52/1 -> Convert31/1
  Register8/1 -> Stage1_ch1-6/3
  Register5/1 -> Stage1_ch1-6/4
  Register13/1 -> Stage1_ch1-6/5
  Register9/1 -> Stage1_ch1-6/6
  Register15/1 -> Stage1_ch1-6/7
  Register16/1 -> Stage1_ch1-6/8
  Register25/1 -> Stage1_ch1-6/9
  Register17/1 -> Stage1_ch1-6/10
  Register27/1 -> Stage1_ch1-6/11
  Register24/1 -> Stage1_ch1-6/12
  Register19/1 -> Stage1_ch7-10/1
  Register31/1 -> Stage1_ch7-10/2
  Register21/1 -> Stage1_ch7-10/3
  Register22/1 -> Stage1_ch7-10/4
  Register40/1 -> Stage1_ch7-10/5
  Register32/1 -> Stage1_ch7-10/6
  Register42/1 -> Stage1_ch7-10/7
  Register39/1 -> Stage1_ch7-10/8
  Convert/1 -> Stage2_ch1-6/1
  Convert2/1 -> Stage2_ch1-6/2
  Convert4/1 -> Stage2_ch1-6/3
  Convert6/1 -> Stage2_ch1-6/4
  Convert8/1 -> Stage2_ch1-6/5
  Convert9/1 -> Stage2_ch1-6/6
  Convert25/1 -> Stage2_ch1-6/7
  Convert26/1 -> Stage2_ch1-6/8
  Convert27/1 -> Stage2_ch1-6/9
  Convert28/1 -> Stage2_ch1-6/10
  Convert29/1 -> Stage2_ch1-6/11
  Convert30/1 -> Stage2_ch1-6/12
  Convert31/1 -> Stage2_ch7-10/1
  Convert32/1 -> Stage2_ch7-10/2
  Convert39/1 -> Stage2_ch7-10/3
  Convert40/1 -> Stage2_ch7-10/4
  Convert41/1 -> Stage2_ch7-10/5
  Convert42/1 -> Stage2_ch7-10/6
  Convert33/1 -> Stage2_ch7-10/7
  Convert34/1 -> Stage2_ch7-10/8
  Stage2_ch1-6/3 -> Shift9/1
  Reinterpret40/1 -> Convert11/1
  Shift11/1 -> Reinterpret40/1
  Stage2_ch1-6/4 -> Shift11/1
  Stage2_ch1-6/6 -> Shift12/1
  Shift12/1 -> Reinterpret42/1
  Reinterpret42/1 -> Convert13/1
  Stage2_ch1-6/5 -> Shift13/1
  Reinterpret41/1 -> Convert12/1
  Shift13/1 -> Reinterpret41/1
  Shift42/1 -> Reinterpret53/1
  Reinterpret53/1 -> Convert43/1
  Stage2_ch1-6/9 -> Shift42/1
  Reinterpret54/1 -> Convert44/1
  Shift15/1 -> Reinterpret54/1
  Stage2_ch1-6/10 -> Shift15/1
  Stage2_ch1-6/8 -> Shift14/1
  Shift14/1 -> Reinterpret44/1
  Reinterpret44/1 -> Convert15/1
  Stage2_ch1-6/7 -> Shift43/1
  Reinterpret43/1 -> Convert14/1
  Shift43/1 -> Reinterpret43/1
  Shift47/1 -> Reinterpret55/1
  Reinterpret55/1 -> Convert45/1
  Stage2_ch1-6/11 -> Shift47/1
  Reinterpret56/1 -> Convert46/1
  Shift44/1 -> Reinterpret56/1
  Stage2_ch1-6/12 -> Shift44/1
  Stage2_ch1-6/14 -> Shift45/1
  Shift45/1 -> Reinterpret58/1
  Reinterpret58/1 -> Convert48/1
  Stage2_ch1-6/13 -> Shift46/1
  Reinterpret57/1 -> Convert47/1
  Shift46/1 -> Reinterpret57/1
  Shift54/1 -> Reinterpret63/1
  Reinterpret63/1 -> Convert53/1
  Stage2_ch7-10/7 -> Shift54/1
  Reinterpret64/1 -> Convert54/1
  Shift51/1 -> Reinterpret64/1
  Stage2_ch7-10/8 -> Shift51/1
  Stage2_ch7-10/10 -> Shift52/1
  Shift52/1 -> Reinterpret66/1
  Reinterpret66/1 -> Convert56/1
  Stage2_ch7-10/9 -> Shift53/1
  Reinterpret65/1 -> Convert55/1
  Shift53/1 -> Reinterpret65/1
  Shift50/1 -> Reinterpret61/1
  Reinterpret61/1 -> Convert51/1
  Stage2_ch7-10/5 -> Shift50/1
  Reinterpret62/1 -> Convert52/1
  Shift49/1 -> Reinterpret62/1
  Stage2_ch7-10/6 -> Shift49/1
  Stage2_ch7-10/4 -> Shift48/1
  Shift48/1 -> Reinterpret60/1
  Reinterpret60/1 -> Convert50/1
  Stage2_ch7-10/3 -> Shift59/1
  Reinterpret59/1 -> Convert49/1
  Shift59/1 -> Reinterpret59/1
  Convert10/1 -> Stage3_ch1-6/1
  Convert11/1 -> Stage3_ch1-6/2
  Convert12/1 -> Stage3_ch1-6/3
  Convert13/1 -> Stage3_ch1-6/4
  Convert14/1 -> Stage3_ch1-6/5
  Convert15/1 -> Stage3_ch1-6/6
  Convert43/1 -> Stage3_ch1-6/7
  Convert44/1 -> Stage3_ch1-6/8
  Convert45/1 -> Stage3_ch1-6/9
  Convert46/1 -> Stage3_ch1-6/10
  Convert47/1 -> Stage3_ch1-6/11
  Convert48/1 -> Stage3_ch1-6/12
  Convert49/1 -> Stage3_ch7-10/1
  Convert50/1 -> Stage3_ch7-10/2
  Convert51/1 -> Stage3_ch7-10/3
  Convert52/1 -> Stage3_ch7-10/4
  Convert53/1 -> Stage3_ch7-10/5
  Convert54/1 -> Stage3_ch7-10/6
  Convert55/1 -> Stage3_ch7-10/7
  Convert56/1 -> Stage3_ch7-10/8
  Stage3_ch1-6/3 -> Shift2/1
  Stage3_ch1-6/4 -> Shift16/1
  Shift16/1 -> Reinterpret45/1
  Reinterpret45/1 -> Convert16/1
  Reinterpret47/1 -> Convert17/1
  Shift17/1 -> Reinterpret47/1
  Stage3_ch1-6/6 -> Shift17/1
  Stage3_ch1-6/5 -> Shift18/1
  Shift18/1 -> Reinterpret46/1
  Reinterpret46/1 -> Convert18/1
  Reinterpret48/1 -> Convert20/1
  Shift20/1 -> Reinterpret48/1
  Stage3_ch1-6/7 -> Shift20/1
  Stage3_ch1-6/8 -> Shift19/1
  Shift19/1 -> Reinterpret49/1
  Reinterpret49/1 -> Convert19/1
  Reinterpret76/1 -> Convert64/1
  Shift63/1 -> Reinterpret76/1
  Stage3_ch1-6/14 -> Shift63/1
  Stage3_ch1-6/13 -> Shift65/1
  Shift65/1 -> Reinterpret75/1
  Reinterpret75/1 -> Convert65/1
  Reinterpret73/1 -> Convert63/1
  Shift62/1 -> Reinterpret73/1
  Stage3_ch1-6/11 -> Shift62/1
  Stage3_ch1-6/12 -> Shift61/1
  Shift61/1 -> Reinterpret74/1
  Reinterpret74/1 -> Convert62/1
  Reinterpret72/1 -> Convert61/1
  Shift60/1 -> Reinterpret72/1
  Stage3_ch1-6/10 -> Shift60/1
  Stage3_ch1-6/9 -> Shift64/1
  Shift64/1 -> Reinterpret71/1
  Reinterpret71/1 -> Convert66/1
  Reinterpret83/1 -> Convert78/1
  Shift76/1 -> Reinterpret83/1
  Stage3_ch7-10/9 -> Shift76/1
  Stage3_ch7-10/10 -> Shift72/1
  Shift72/1 -> Reinterpret84/1
  Reinterpret84/1 -> Convert73/1
  Reinterpret82/1 -> Convert70/1
  Shift69/1 -> Reinterpret82/1
  Stage3_ch7-10/8 -> Shift69/1
  Stage3_ch7-10/7 -> Shift71/1
  Shift71/1 -> Reinterpret81/1
  Reinterpret81/1 -> Convert71/1
  Reinterpret79/1 -> Convert69/1
  Shift68/1 -> Reinterpret79/1
  Stage3_ch7-10/5 -> Shift68/1
  Stage3_ch7-10/6 -> Shift67/1
  Shift67/1 -> Reinterpret80/1
  Reinterpret80/1 -> Convert68/1
  Reinterpret78/1 -> Convert67/1
  Shift66/1 -> Reinterpret78/1
  Stage3_ch7-10/4 -> Shift66/1
  Stage3_ch7-10/3 -> Shift70/1
  Shift70/1 -> Reinterpret77/1
  Reinterpret77/1 -> Convert72/1
  Convert3/1 -> Stage4_ch1-6/1
  Convert16/1 -> Stage4_ch1-6/2
  Convert18/1 -> Stage4_ch1-6/3
  Convert17/1 -> Stage4_ch1-6/4
  Convert20/1 -> Stage4_ch1-6/5
  Convert19/1 -> Stage4_ch1-6/6
  Convert66/1 -> Stage4_ch1-6/7
  Convert61/1 -> Stage4_ch1-6/8
  Convert63/1 -> Stage4_ch1-6/9
  Convert62/1 -> Stage4_ch1-6/10
  Convert65/1 -> Stage4_ch1-6/11
  Convert64/1 -> Stage4_ch1-6/12
  Convert72/1 -> Stage4_ch7-10/1
  Convert67/1 -> Stage4_ch7-10/2
  Convert69/1 -> Stage4_ch7-10/3
  Convert68/1 -> Stage4_ch7-10/4
  Convert71/1 -> Stage4_ch7-10/5
  Convert70/1 -> Stage4_ch7-10/6
  Convert78/1 -> Stage4_ch7-10/7
  Convert73/1 -> Stage4_ch7-10/8
  Stage4_ch1-6/3 -> Shift4/1
  Stage4_ch1-6/4 -> Shift21/1
  Shift21/1 -> Reinterpret7/1
  Reinterpret7/1 -> Convert7/1
  Reinterpret9/1 -> Convert22/1
  Shift22/1 -> Reinterpret9/1
  Stage4_ch1-6/6 -> Shift22/1
  Stage4_ch1-6/5 -> Shift23/1
  Shift23/1 -> Reinterpret8/1
  Reinterpret8/1 -> Convert21/1
  Reinterpret10/1 -> Convert23/1
  Shift25/1 -> Reinterpret10/1
  Stage4_ch1-6/7 -> Shift25/1
  Stage4_ch1-6/8 -> Shift24/1
  Shift24/1 -> Reinterpret11/1
  Reinterpret11/1 -> Convert24/1
  Reinterpret90/1 -> Convert82/1
  Shift81/1 -> Reinterpret90/1
  Stage4_ch1-6/14 -> Shift81/1
  Stage4_ch1-6/13 -> Shift82/1
  Shift82/1 -> Reinterpret89/1
  Reinterpret89/1 -> Convert81/1
  Reinterpret93/1 -> Convert79/1
  Shift80/1 -> Reinterpret93/1
  Stage4_ch1-6/11 -> Shift80/1
  Stage4_ch1-6/12 -> Shift79/1
  Shift79/1 -> Reinterpret94/1
  Reinterpret94/1 -> Convert80/1
  Reinterpret92/1 -> Convert84/1
  Shift78/1 -> Reinterpret92/1
  Stage4_ch1-6/10 -> Shift78/1
  Stage4_ch1-6/9 -> Shift83/1
  Shift83/1 -> Reinterpret91/1
  Reinterpret91/1 -> Convert83/1
  Reinterpret103/1 -> Convert95/1
  Shift95/1 -> Reinterpret103/1
  Stage4_ch7-10/9 -> Shift95/1
  Stage4_ch7-10/10 -> Shift90/1
  Shift90/1 -> Reinterpret104/1
  Reinterpret104/1 -> Convert96/1
  Reinterpret96/1 -> Convert88/1
  Shift87/1 -> Reinterpret96/1
  Stage4_ch7-10/8 -> Shift87/1
  Stage4_ch7-10/7 -> Shift88/1
  Shift88/1 -> Reinterpret95/1
  Reinterpret95/1 -> Convert87/1
  Reinterpret99/1 -> Convert85/1
  Shift86/1 -> Reinterpret99/1
  Stage4_ch7-10/5 -> Shift86/1
  Stage4_ch7-10/6 -> Shift85/1
  Shift85/1 -> Reinterpret101/1
  Reinterpret101/1 -> Convert86/1
  Reinterpret98/1 -> Convert90/1
  Shift84/1 -> Reinterpret98/1
  Stage4_ch7-10/4 -> Shift84/1
  Stage4_ch7-10/3 -> Shift89/1
  Shift89/1 -> Reinterpret97/1
  Reinterpret97/1 -> Convert89/1
  Convert5/1 -> Stage5_ch1-6/1
  Convert7/1 -> Stage5_ch1-6/2
  Convert21/1 -> Stage5_ch1-6/3
  Convert22/1 -> Stage5_ch1-6/4
  Convert23/1 -> Stage5_ch1-6/5
  Convert24/1 -> Stage5_ch1-6/6
  Convert83/1 -> Stage5_ch1-6/7
  Convert84/1 -> Stage5_ch1-6/8
  Convert79/1 -> Stage5_ch1-6/9
  Convert80/1 -> Stage5_ch1-6/10
  Convert81/1 -> Stage5_ch1-6/11
  Convert82/1 -> Stage5_ch1-6/12
  Convert89/1 -> Stage5_ch7-10/1
  Convert90/1 -> Stage5_ch7-10/2
  Convert85/1 -> Stage5_ch7-10/3
  Convert86/1 -> Stage5_ch7-10/4
  Convert87/1 -> Stage5_ch7-10/5
  Convert88/1 -> Stage5_ch7-10/6
  Convert95/1 -> Stage5_ch7-10/7
  Convert96/1 -> Stage5_ch7-10/8
  Stage1_ch1-6/1 -> Terminator12/1
  Stage1_ch1-6/2 -> Terminator13/1
  Stage2_ch1-6/2 -> Terminator18/1
  Stage2_ch1-6/1 -> Terminator10/1
  Stage3_ch1-6/1 -> Terminator20/1
  Stage3_ch1-6/2 -> Terminator21/1
  Stage4_ch1-6/2 -> Terminator23/1
  Stage4_ch1-6/1 -> Terminator22/1
  Stage5_ch1-6/1 -> Terminator24/1
  Stage5_ch1-6/2 -> Terminator26/1
  Stage5_ch1-6/3 -> Reinterpret2/1
  Stage5_ch1-6/4 -> Reinterpret1/1
  Stage5_ch1-6/6 -> Reinterpret3/1
  Stage5_ch1-6/5 -> Reinterpret4/1
  Reinterpret2/1 -> BitBasher3/1
  Reinterpret1/1 -> BitBasher3/2
  Reinterpret4/1 -> BitBasher4/1
  Reinterpret3/1 -> BitBasher4/2
  Stage5_ch1-6/7 -> Reinterpret6/1
  Stage5_ch1-6/8 -> Reinterpret5/1
  Stage5_ch1-6/14 -> Reinterpret111/1
  Stage5_ch1-6/13 -> Reinterpret112/1
  Stage5_ch1-6/11 -> Reinterpret110/1
  Stage5_ch1-6/12 -> Reinterpret109/1
  Stage5_ch1-6/10 -> Reinterpret107/1
  Stage5_ch1-6/9 -> Reinterpret108/1
  Stage5_ch7-10/9 -> Reinterpret115/1
  Stage5_ch7-10/10 -> Reinterpret114/1
  Stage5_ch7-10/8 -> Reinterpret123/1
  Stage5_ch7-10/7 -> Reinterpret124/1
  Stage5_ch7-10/5 -> Reinterpret122/1
  Stage5_ch7-10/6 -> Reinterpret121/1
  Stage5_ch7-10/4 -> Reinterpret113/1
  Stage5_ch7-10/3 -> Reinterpret120/1
  Stage1_ch7-10/2 -> Terminator27/1
  Stage1_ch7-10/1 -> Terminator14/1
  Stage2_ch7-10/1 -> Terminator29/1
  Stage2_ch7-10/2 -> Terminator30/1
  Stage3_ch7-10/2 -> Terminator32/1
  Stage3_ch7-10/1 -> Terminator31/1
  Stage4_ch7-10/1 -> Terminator33/1
  Stage4_ch7-10/2 -> Terminator34/1
  Stage5_ch7-10/2 -> Terminator37/1
  Stage5_ch7-10/1 -> Terminator35/1
  Reinterpret6/1 -> BitBasher5/1
  Reinterpret5/1 -> BitBasher5/2
  Reinterpret108/1 -> BitBasher6/1
  Reinterpret107/1 -> BitBasher6/2
  Reinterpret110/1 -> BitBasher7/1
  Reinterpret109/1 -> BitBasher7/2
  Reinterpret112/1 -> BitBasher8/1
  Reinterpret111/1 -> BitBasher8/2
  pipeline12/1(q) -> Mux3/2
  pipeline1/1(q) -> Mux3/3
  pipeline2/1(q) -> Mux3/5
  pipeline3/1(q) -> Mux3/4
  pipeline5/1(q) -> Mux3/6
  pipeline4/1(q) -> Mux3/7
  pipeline9/1(q) -> Mux3/10
  pipeline8/1(q) -> Mux3/11
  pipeline6/1(q) -> Mux3/9
  pipeline7/1(q) -> Mux3/8
  Constant7/1 -> Mux3/17, Mux3/16, Mux3/15, Mux3/12, Mux3/13, Mux3/14
  Reinterpret114/1 -> BitBasher12/2
  Reinterpret115/1 -> BitBasher12/1
  Reinterpret123/1 -> BitBasher11/2
  Reinterpret124/1 -> BitBasher11/1
  Reinterpret121/1 -> BitBasher10/2
  Reinterpret122/1 -> BitBasher10/1
  Reinterpret113/1 -> BitBasher9/2
  Reinterpret120/1 -> BitBasher9/1
  [channelIdx] -> Mux3/1
  Mux3/1 -> Mux4/4
  BitBasher3/1 -> pipeline12/1(d)
  BitBasher4/1 -> pipeline1/1(d)
  BitBasher5/1 -> pipeline3/1(d)
  BitBasher6/1 -> pipeline2/1(d)
  BitBasher7/1 -> pipeline5/1(d)
  BitBasher8/1 -> pipeline4/1(d)
  BitBasher9/1 -> pipeline7/1(d)
  BitBasher10/1 -> pipeline6/1(d)
  BitBasher11/1 -> pipeline9/1(d)
  BitBasher12/1 -> pipeline8/1(d)
  gbe0/6(rx_data) -> Register47/1
  [end_pkt] -> gbe0/6(tx_end_of_frame)
  [reset_gbe0] -> gbe0/1(rst)
  gbe0/2(led_rx) -> Terminator36/1
  gbe0/4(tx_afull) -> Terminator49/1
  gbe0/12(rx_overrun) -> Terminator40/1
  gbe0/3(led_tx) -> Terminator25/1
  Delay1/1 -> gbe0/8(rx_overrun_ack)
  Constant4/1 -> dest_ip/1(sim_1)
  Constant8/1 -> dest_port/1(sim_1)
  gbe0/5(tx_overflow) -> Terminator48/1
  gbe0/11(rx_bad_frame) -> Delay1/1
  gbe0/9(rx_source_port) -> Terminator43/1
  gbe0/8(rx_source_ip) -> Terminator45/1
  dest_port/1(in_reg) -> gbe0/5(tx_dest_port)
  Constant9/1 -> gbe0/7(rx_ack)
  [reset_gbe0] -> gbe0/9(debug_rst)
  dest_ip/1(in_reg) -> gbe0/4(tx_dest_ip)
  Logical3/1 -> [eth_valid]
  Register44/1 -> led3/1
  led3/1 -> Terminator38/1
  [end_pkt] -> Register30/1
  pulse_ext2/1(out) -> Register44/1
  Register30/1 -> pulse_ext2/1(in)
  Register29/1 -> gbe0/2(tx_data)
  Register28/1 -> gbe0/3(tx_valid)
  gbe0/1(led_up) -> [gbe0_up]
  Register45/1 -> led1/1
  led1/1 -> Terminator6/1
  [gbe0_up] -> Register45/1
  Slice2/1 -> [reset_gbe0]
  reset_gbe0/1(in_reg) -> Register46/1
  Register46/1 -> Slice2/1
  Constant1/1 -> reset_gbe0/1(sim_1)
  Register47/1 -> Mux1/3
  Reinterpret25/1 -> Mux1/1
  Mux1/1 -> Relational1/2
  Constant5/1 -> Mux1/2
  Constant6/1 -> Relational1/1
  Pulse Generator/1 -> pps/1
  Relational1/1 -> [trigger_1pps]
  Counter4/1 -> Slice5/1
  [reset_pktcnt] -> Counter4/1
  pps/1 -> edge_detect1/1(in)
  Slice5/1 -> Logical1/3, Inverter2/1
  edge_detect1/1(out) -> Logical1/2
  Register48/1 -> Reinterpret25/1
  Slice4/1 -> Logical1/1, edge_detect2/1(in), Logical8/1
  snap_adc/11(c3) -> Terminator15/1
  snap_adc/12(c4) -> Terminator16/1
  gbe0/10(rx_end_of_frame) -> Terminator46/1
  gbe0/7(rx_valid) -> Register48/1
  Counter1/1 -> Slice3/1
  Logical9/1 -> Counter4/2
  [trigger_1pps] -> Logical9/1
  Inverter2/1 -> Logical9/2
  Logical1/1 -> Counter1/2
  Slice3/1 -> Logical8/2
  edge_detect2/1(out) -> Counter1/1
  Logical8/1 -> Delay4/1, edge_detect9/1(in)
